simulink model "Test2_2"  (R2021a)
(part 1 of 3)
settings: Solver=FixedStepAuto  StartTime=0  StopTime=0.2  FixedStep=0.2  RelTol=1e-3
libraries: spsDistributedParametersLineLib x212, spsThreePhaseSeriesRLCLoadLib x70, spsThreePhaseVIMeasurementLib x8, spsGroundLib x1, spsThreePhaseSourceLib x1, spsSeriesRLCBranchLib x1, spspowerguiLib x1
settings Model: Creator=Admin  LastModifiedBy=Admin

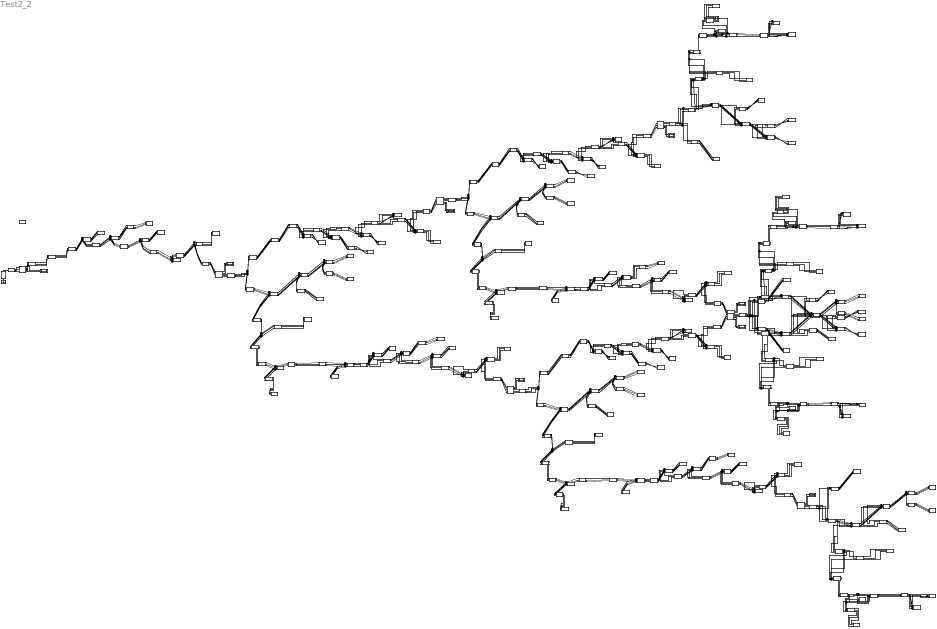
== system Test2_2 ==
  Ground : spsGroundLib/Ground  LConnTagsString=a
  Line 1 : spsDistributedParametersLineLib/Distributed Parameters Line  Phases=3  Length=1.11  Frequency=50  Resistance=[0.502970710632245 0.0486237908083191 0.0486712220507153;0.0486237908083191 0.502875844822084 0.0486237934466192;0.0486712220507153 0.0486237934466192 0.502970710632245]  Inductance=[0.00286900545038753 0.00133270803418135 0.00132951476746136;0.00133270803418135 0.00286931445999602 0.00133799988507366;0.00132951476746136 0.00133799988507366 0.00286900545038753]  Capacitance=[8.11484299003193e-09 -1.94249816214699e-09 -1.86930692621136e-09;-1.94249816214699e-09 8.0425699231653e-09 -1.98049571960044e-09;-1.86930692621136e-09 -1.98049571960044e-09 8.13337738722527e-09]  x1=[235.740627449821 9842.13785797111 9841.50657979125;314.159265358979 314.159265358979 314.159265358979;1.08127877463144 2.25146816148109 -2.46064601505037]  x2=[235.740963564487 9842.14706191756 9841.51580387368;314.159265358979 314.159265358979 314.159265358979;1.08127828242004 2.25146728367899 -2.46064690041362]  x3=[0.20667213359049 25.036273858011 25.2268910022424;314.159265358979 314.159265358979 314.159265358979;1.079589872229 2.25010012848936 -2.46201559089723]  x4=[0.206672133614643 25.0362738655198 25.2268910099133;314.159265358979 314.159265358979 314.159265358979;1.08127828238506 2.25146728367861 -2.46064690041429]  x5=5.37516004033389e-06  V1=ones(3,3)  V2=ones(3,3)  I1=ones(3,3)  I2=ones(3,3)  nHarmo=1  Measurements=None  Decoupling=off  VsMag0=0  VrMag0=0  VsAngle0=0  VrAngle0=0  IsMag0=0  IrMag0=0  IsAngle0=0  IrAngle0=0
      settings: SourceProductBaseCode=PS
  Line 10 : spsDistributedParametersLineLib/Distributed Parameters Line  Phases=3  Length=0.02  Frequency=50  Resistance=[0.646656091154803 0.0486237908083191 0.0486712220507153;0.0486237908083191 0.646561225344642 0.0486237934466192;0.0486712220507153 0.0486237934466192 0.646656091154803]  Inductance=[0.00282448912315926 0.00133270803418135 0.00132951476746136;0.00133270803418135 0.00282479813276775 0.00133799988507366;0.00132951476746136 0.00133799988507366 0.00282448912315926]  Capacitance=[7.89543174552926e-09 -1.85986777702161e-09 -1.7901190036642e-09;-1.85986777702161e-09 7.82540023894543e-09 -1.8957321828871e-09;-1.7901190036642e-09 -1.8957321828871e-09 7.91264394645417e-09]  x1=[131.78014733242 9843.57612220075 9843.09391339889;314.159265358979 314.159265358979 314.159265358979;1.07009614058309 2.25918230682552 -2.45295604852824]  x2=[131.780254208923 9843.54629581266 9843.0641121035;314.159265358979 314.159265358979 314.159265358979;1.07009786039608 2.25918056584775 -2.45295777590887]  x3=[0.121897583666128 22.8143812661449 23.0053055695837;314.159265358979 314.159265358979 314.159265358979;1.06824602708052 2.27345686414031 -2.43881138170621]  x4=[0.108540682306908 27.2903157642653 27.4816698646594;314.159265358979 314.159265358979 314.159265358979;1.07214379525045 2.24722551403408 -2.46482021330641]  x5=9.5829454252223e-08  V1=ones(3,3)  V2=ones(3,3)  I1=ones(3,3)  I2=ones(3,3)  nHarmo=1  Measurements=None  Decoupling=off  VsMag0=0  VrMag0=0  VsAngle0=0  VrAngle0=0  IsMag0=0  IrMag0=0  IsAngle0=0  IrAngle0=0
      settings: SourceProductBaseCode=PS
  Line 100 : spsDistributedParametersLineLib/Distributed Parameters Line  Phases=3  Length=0.12001  Frequency=50  Resistance=[0.646656091154803 0.0486237908083191 0.0486712220507153;0.0486237908083191 0.646561225344642 0.0486237934466192;0.0486712220507153 0.0486237934466192 0.646656091154803]  Inductance=[0.00282448912315926 0.00133270803418135 0.00132951476746136;0.00133270803418135 0.00282479813276775 0.00133799988507366;0.00132951476746136 0.00133799988507366 0.00282448912315926]  Capacitance=[7.89543174552926e-09 -1.85986777702161e-09 -1.7901190036642e-09;-1.85986777702161e-09 7.82540023894543e-09 -1.8957321828871e-09;-1.7901190036642e-09 -1.8957321828871e-09 7.91264394645417e-09]  x1=[132.251183868736 9822.51156326851 9822.6881155278;314.159265358979 314.159265358979 314.159265358979;1.0139776910405 -0.191624464327191 -1.76260238554906]  x2=[132.251379700384 9822.48352849832 9822.66014018258;314.159265358979 314.159265358979 314.159265358979;1.01397817548804 -0.191624813198916 -1.76260272547254]  x3=[0.116233256836359 24.7295911584912 24.9218766604658;314.159265358979 314.159265358979 314.159265358979;1.00798240761241 -0.185214983818316 -1.75624522525873]  x4=[0.115021145519369 25.2589468937937 25.4514391532114;314.159265358979 314.159265358979 314.159265358979;1.01985503692047 -0.198041980394282 -1.76896977112499]  x5=5.75024640240464e-07  V1=ones(3,3)  V2=ones(3,3)  I1=ones(3,3)  I2=ones(3,3)  nHarmo=1  Measurements=None  Decoupling=off  VsMag0=0  VrMag0=0  VsAngle0=0  VrAngle0=0  IsMag0=0  IrMag0=0  IsAngle0=0  IrAngle0=0
      settings: SourceProductBaseCode=PS
  Line 101 : spsDistributedParametersLineLib/Distributed Parameters Line  Phases=3  Length=0.82  Frequency=50  Resistance=[0.646656091154803 0.0486237908083191 0.0486712220507153;0.0486237908083191 0.646561225344642 0.0486237934466192;0.0486712220507153 0.0486237934466192 0.646656091154803]  Inductance=[0.00282448912315926 0.00133270803418135 0.00132951476746136;0.00133270803418135 0.00282479813276775 0.00133799988507366;0.00132951476746136 0.00133799988507366 0.00282448912315926]  Capacitance=[7.89543174552926e-09 -1.85986777702161e-09 -1.7901190036642e-09;-1.85986777702161e-09 7.82540023894543e-09 -1.8957321828871e-09;-1.7901190036642e-09 -1.8957321828871e-09 7.91264394645417e-09]  x1=[132.251183868736 9822.51156326851 9822.6881155278;314.159265358979 314.159265358979 314.159265358979;1.01292400621019 -0.192461547720951 -1.76344026578694]  x2=[132.254706380519 9821.98923988506 9822.16651105881;314.159265358979 314.159265358979 314.159265358979;1.01294030353769 -0.192482605604276 -1.76346112432621]  x3=[0.117790876870439 24.1120519373959 24.3038670356319;314.159265358979 314.159265358979 314.159265358979;0.99917348478268 -0.182323882366389 -1.75339911559519]  x4=[0.113404341728002 25.8369348193095 26.0292631540775;314.159265358979 314.159265358979 314.159265358979;1.02596467431606 -0.202890909757443 -1.77378526157166]  x5=3.92900762434114e-06  V1=ones(3,3)  V2=ones(3,3)  I1=ones(3,3)  I2=ones(3,3)  nHarmo=1  Measurements=None  Decoupling=off  VsMag0=0  VrMag0=0  VsAngle0=0  VrAngle0=0  IsMag0=0  IrMag0=0  IsAngle0=0  IrAngle0=0
      settings: SourceProductBaseCode=PS
  Line 102 : spsDistributedParametersLineLib/Distributed Parameters Line  Phases=3  Length=1.11  Frequency=50  Resistance=[0.646656091154803 0.0486237908083191 0.0486712220507153;0.0486237908083191 0.646561225344642 0.0486237934466192;0.0486712220507153 0.0486237934466192 0.646656091154803]  Inductance=[0.00282448912315926 0.00133270803418135 0.00132951476746136;0.00133270803418135 0.00282479813276775 0.00133799988507366;0.00132951476746136 0.00133799988507366 0.00282448912315926]  Capacitance=[7.89543174552926e-09 -1.85986777702161e-09 -1.7901190036642e-09;-1.85986777702161e-09 7.82540023894543e-09 -1.8957321828871e-09;-1.7901190036642e-09 -1.8957321828871e-09 7.91264394645417e-09]  x1=[132.22110603618 9826.55451502118 9826.72616066843;314.159265358979 314.159265358979 314.159265358979;1.01234684176435 -0.192590861949341 -1.76357146343656]  x2=[132.238781069031 9824.24966881277 9824.42365326744;314.159265358979 314.159265358979 314.159265358979;1.01243597193449 -0.192738058848091 -1.76371774540788]  x3=[0.124232108565467 21.7752977626428 21.9664339216675;314.159265358979 314.159265358979 314.159265358979;0.966849600717489 -0.177729233813201 -1.7489636968201]  x4=[0.107137659712284 28.1752500802333 28.3680257860225;314.159265358979 314.159265358979 314.159265358979;1.06340115095006 -0.205384100987335 -1.77619162891763]  x5=5.31853471099837e-06  V1=ones(3,3)  V2=ones(3,3)  I1=ones(3,3)  I2=ones(3,3)  nHarmo=1  Measurements=None  Decoupling=off  VsMag0=0  VrMag0=0  VsAngle0=0  VrAngle0=0  IsMag0=0  IrMag0=0  IsAngle0=0  IrAngle0=0
      settings: SourceProductBaseCode=PS
  Line 103 : spsDistributedParametersLineLib/Distributed Parameters Line  Phases=3  Length=0.20999  Frequency=50  Resistance=[0.646656091154803 0.0486237908083191 0.0486712220507153;0.0486237908083191 0.646561225344642 0.0486237934466192;0.0486712220507153 0.0486237934466192 0.646656091154803]  Inductance=[0.00282448912315926 0.00133270803418135 0.00132951476746136;0.00133270803418135 0.00282479813276775 0.00133799988507366;0.00132951476746136 0.00133799988507366 0.00282448912315926]  Capacitance=[7.89543174552926e-09 -1.85986777702161e-09 -1.7901190036642e-09;-1.85986777702161e-09 7.82540023894543e-09 -1.8957321828871e-09;-1.7901190036642e-09 -1.8957321828871e-09 7.91264394645417e-09]  x1=[132.22110603618 9826.55451502118 9826.72616066843;314.159265358979 314.159265358979 314.159265358979;1.01370161380985 -0.191514584537925 -1.76249416148526]  x2=[132.220703418741 9826.60479396299 9826.77613530937;314.159265358979 314.159265358979 314.159265358979;1.01370438274641 -0.191521096517127 -1.76250067247797]  x3=[0.11604976886815 25.0066881755724 25.1992168467069;314.159265358979 314.159265358979 314.159265358979;1.02480830153253 -0.212018461817681 -1.78284780104421]  x4=[0.11515209619338 25.0068429368372 25.1990818745629;314.159265358979 314.159265358979 314.159265358979;1.00219378168083 -0.171268482071947 -1.74239830051209]  x5=1.00616135492121e-06  V1=ones(3,3)  V2=ones(3,3)  I1=ones(3,3)  I2=ones(3,3)  nHarmo=1  Measurements=None  Decoupling=off  VsMag0=0  VrMag0=0  VsAngle0=0  VrAngle0=0  IsMag0=0  IrMag0=0  IsAngle0=0  IrAngle0=0
      settings: SourceProductBaseCode=PS
  Line 104 : spsDistributedParametersLineLib/Distributed Parameters Line  Phases=3  Length=0.23001  Frequency=50  Resistance=[0.476003738225748 0.351747138225748 0.351747138225748;0.351747138225748 0.476003738225748 0.351747138225748;0.351747138225748 0.351747138225748 0.476003738225748]  Inductance=[0.000705954362986426 0.000459934243504405 0.000459934243504405;0.000459934243504405 0.000705954362986426 0.000459934243504405;0.000459934243504405 0.000459934243504405 0.000705954362986426]  Capacitance=[5.7561313269996e-07 -1.37543883484145e-07 -1.37543912800485e-07;-1.37543883484145e-07 5.75613027339387e-07 -1.37543875208088e-07;-1.37543912800485e-07 -1.37543875208088e-07 5.75613005057695e-07]  x1=[4.47229783792521 9827.65587276305 9828.6527718167;314.159265358979 314.159265358979 314.159265358979;1.27259155336982 -0.110574029317674 -1.68141113561575]  x2=[4.47230354283643 9827.66037438348 9828.65727389307;314.159265358979 314.159265358979 314.159265358979;1.27258860764781 -0.110574765724932 -1.6814118720229]  x3=[0.0606364727518491 528.513670062988 528.567240688046;314.159265358979 314.159265358979 314.159265358979;1.27099282696656 -0.111531535342372 -1.68236864156729]  x4=[0.0606364726692423 528.513670156436 528.567240781746;314.159265358979 314.159265358979 314.159265358979;1.27258860804999 -0.110574765725967 -1.68141187202331]  x5=5.08421409621804e-06  V1=ones(3,3)  V2=ones(3,3)  I1=ones(3,3)  I2=ones(3,3)  nHarmo=1  Measurements=None  Decoupling=off  VsMag0=0  VrMag0=0  VsAngle0=0  VrAngle0=0  IsMag0=0  IrMag0=0  IsAngle0=0  IrAngle0=0
      settings: SourceProductBaseCode=PS
  Line 105 : spsDistributedParametersLineLib/Distributed Parameters Line  Phases=3  Length=0.28003  Frequency=50  Resistance=[0.646656091154803 0.0486237908083191 0.0486712220507153;0.0486237908083191 0.646561225344642 0.0486237934466192;0.0486712220507153 0.0486237934466192 0.646656091154803]  Inductance=[0.00282448912315926 0.00133270803418135 0.00132951476746136;0.00133270803418135 0.00282479813276775 0.00133799988507366;0.00132951476746136 0.00133799988507366 0.00282448912315926]  Capacitance=[7.89543174552926e-09 -1.85986777702161e-09 -1.7901190036642e-09;-1.85986777702161e-09 7.82540023894543e-09 -1.8957321828871e-09;-1.7901190036642e-09 -1.8957321828871e-09 7.91264394645417e-09]  x1=[131.783203312388 9842.18139381324 9841.69855997394;314.159265358979 314.159265358979 314.159265358979;1.06980400384549 2.25872965727568 -2.45340823480742]  x2=[131.783260319828 9842.18412601891 9841.70129695104;314.159265358979 314.159265358979 314.159265358979;1.06980381572691 2.25872930408743 -2.45340859096022]  x3=[0.115206681531441 25.0392814649209 25.2302987105999;314.159265358979 314.159265358979 314.159265358979;1.06856559283218 2.25773315191792 -2.45440562091191]  x4=[0.115207403330286 25.0392810388126 25.2302991433172;314.159265358979 314.159265358979 314.159265358979;1.07062067597059 2.25939089977307 -2.45274643363381]  x5=1.3417561037125e-06  V1=ones(3,3)  V2=ones(3,3)  I1=ones(3,3)  I2=ones(3,3)  nHarmo=1  Measurements=None  Decoupling=off  VsMag0=0  VrMag0=0  VsAngle0=0  VrAngle0=0  IsMag0=0  IrMag0=0  IsAngle0=0  IrAngle0=0
      settings: SourceProductBaseCode=PS
  Line 106 : spsDistributedParametersLineLib/Distributed Parameters Line  Phases=3  Length=0.24001  Frequency=50  Resistance=[0.646656091154803 0.0486237908083191 0.0486712220507153;0.0486237908083191 0.646561225344642 0.0486237934466192;0.0486712220507153 0.0486237934466192 0.646656091154803]  Inductance=[0.00282448912315926 0.00133270803418135 0.00132951476746136;0.00133270803418135 0.00282479813276775 0.00133799988507366;0.00132951476746136 0.00133799988507366 0.00282448912315926]  Capacitance=[7.89543174552926e-09 -1.85986777702161e-09 -1.7901190036642e-09;-1.85986777702161e-09 7.82540023894543e-09 -1.8957321828871e-09;-1.7901190036642e-09 -1.8957321828871e-09 7.91264394645417e-09]  x1=[132.202684239385 9826.99999536629 9827.16500331793;314.159265358979 314.159265358979 314.159265358979;1.01370346118121 -0.19151111998988 -1.76249021593862]  x2=[132.221106036175 9826.55451502137 9826.72616066862;314.159265358979 314.159265358979 314.159265358979;1.01365642513771 -0.191550483970015 -1.76253009509107]  x3=[0.126648550680777 21.7742149177941 21.9706116888815;314.159265358979 314.159265358979 314.159265358979;0.666612685174768 -0.198929797050631 -1.77234979456121]  x4=[0.120050164818543 28.2292431455141 28.4184691523611;314.159265358979 314.159265358979 314.159265358979;1.38032867226061 -0.186077938239135 -1.75515779675378]  x5=1.1500013657538e-06  V1=ones(3,3)  V2=ones(3,3)  I1=ones(3,3)  I2=ones(3,3)  nHarmo=1  Measurements=None  Decoupling=off  VsMag0=0  VrMag0=0  VsAngle0=0  VrAngle0=0  IsMag0=0  IrMag0=0  IsAngle0=0  IrAngle0=0
      settings: SourceProductBaseCode=PS
  Line 107 : spsDistributedParametersLineLib/Distributed Parameters Line  Phases=3  Length=0.03  Frequency=50  Resistance=[0.476003738225748 0.351747138225748 0.351747138225748;0.351747138225748 0.476003738225748 0.351747138225748;0.351747138225748 0.351747138225748 0.476003738225748]  Inductance=[0.000705954362986426 0.000459934243504405 0.000459934243504405;0.000459934243504405 0.000705954362986426 0.000459934243504405;0.000459934243504405 0.000459934243504405 0.000705954362986426]  Capacitance=[5.7561313269996e-07 -1.37543883484145e-07 -1.37543912800485e-07;-1.37543883484145e-07 5.75613027339387e-07 -1.37543875208088e-07;-1.37543912800485e-07 -1.37543875208088e-07 5.75613005057695e-07]  x1=[4.54470074903476 9824.69388809356 9825.69440909867;314.159265358979 314.159265358979 314.159265358979;1.2803214431057 -0.109972978030824 -1.68080889003995]  x2=[4.54470136219724 9824.6940440882 9825.69456555461;314.159265358979 314.159265358979 314.159265358979;1.28031883175789 -0.109973003530376 -1.68080891566607]  x3=[0.0616594487826835 528.884637500599 528.938393425842;314.159265358979 314.159265358979 314.159265358979;1.2755352456308 -0.110162497062282 -1.68099896514834]  x4=[0.0618747640776966 528.884574036237 528.938456879702;314.159265358979 314.159265358979 314.159265358979;1.28488039234838 -0.109908329382083 -1.68074368546453]  x5=6.63129528657629e-07  V1=ones(3,3)  V2=ones(3,3)  I1=ones(3,3)  I2=ones(3,3)  nHarmo=1  Measurements=None  Decoupling=off  VsMag0=0  VrMag0=0  VsAngle0=0  VrAngle0=0  IsMag0=0  IrMag0=0  IsAngle0=0  IrAngle0=0
      settings: SourceProductBaseCode=PS
  Line 108 : spsDistributedParametersLineLib/Distributed Parameters Line  Phases=3  Length=0.02  Frequency=50  Resistance=[0.646656091154803 0.0486237908083191 0.0486712220507153;0.0486237908083191 0.646561225344642 0.0486237934466192;0.0486712220507153 0.0486237934466192 0.646656091154803]  Inductance=[0.00282448912315926 0.00133270803418135 0.00132951476746136;0.00133270803418135 0.00282479813276775 0.00133799988507366;0.00132951476746136 0.00133799988507366 0.00282448912315926]  Capacitance=[7.89543174552926e-09 -1.85986777702161e-09 -1.7901190036642e-09;-1.85986777702161e-09 7.82540023894543e-09 -1.8957321828871e-09;-1.7901190036642e-09 -1.8957321828871e-09 7.91264394645417e-09]  x1=[132.202684239385 9826.99999536629 9827.16500331793;314.159265358979 314.159265358979 314.159265358979;1.01403463905449 -0.191248020920663 -1.76222686641772]  x2=[132.202716264605 9826.99502778241 9827.16004186565;314.159265358979 314.159265358979 314.159265358979;1.01403480645883 -0.191248234329926 -1.76222707785219]  x3=[0.116469758306098 24.6662306908165 24.8586235131847;314.159265358979 314.159265358979 314.159265358979;1.00929302677894 -0.187472612867995 -1.75848399497354]  x4=[0.114709498477322 25.3502366672254 25.5428305195539;314.159265358979 314.159265358979 314.159265358979;1.01881884545757 -0.194945364619181 -1.76589330632791]  x5=9.5829454252223e-08  V1=ones(3,3)  V2=ones(3,3)  I1=ones(3,3)  I2=ones(3,3)  nHarmo=1  Measurements=None  Decoupling=off  VsMag0=0  VrMag0=0  VsAngle0=0  VrAngle0=0  IsMag0=0  IrMag0=0  IsAngle0=0  IrAngle0=0
      settings: SourceProductBaseCode=PS
  Line 109 : spsDistributedParametersLineLib/Distributed Parameters Line  Phases=3  Length=0.5  Frequency=50  Resistance=[0.646656091154803 0.0486237908083191 0.0486712220507153;0.0486237908083191 0.646561225344642 0.0486237934466192;0.0486712220507153 0.0486237934466192 0.646656091154803]  Inductance=[0.00282448912315926 0.00133270803418135 0.00132951476746136;0.00133270803418135 0.00282479813276775 0.00133799988507366;0.00132951476746136 0.00133799988507366 0.00282448912315926]  Capacitance=[7.89543174552926e-09 -1.85986777702161e-09 -1.7901190036642e-09;-1.85986777702161e-09 7.82540023894543e-09 -1.8957321828871e-09;-1.7901190036642e-09 -1.8957321828871e-09 7.91264394645417e-09]  x1=[132.163450439569 9828.04961373003 9828.20063661273;314.159265358979 314.159265358979 314.159265358979;1.0134061317629 -0.191734356431076 -1.76271272153296]  x2=[132.202684239385 9826.99999536629 9827.16500331793;314.159265358979 314.159265358979 314.159265358979;1.01331210199175 -0.191822029162216 -1.76280142107447]  x3=[0.127642642019091 21.4277763025714 21.6237569851515;314.159265358979 314.159265358979 314.159265358979;0.663833530086098 -0.195610038536538 -1.76910978339631]  x4=[0.119417037015529 28.5638731580296 28.7529094890207;314.159265358979 314.159265358979 314.159265358979;1.38732746175765 -0.189426988396327 -1.75850389104283]  x5=2.39573635630557e-06  V1=ones(3,3)  V2=ones(3,3)  I1=ones(3,3)  I2=ones(3,3)  nHarmo=1  Measurements=None  Decoupling=off  VsMag0=0  VrMag0=0  VsAngle0=0  VrAngle0=0  IsMag0=0  IrMag0=0  IsAngle0=0  IrAngle0=0
      settings: SourceProductBaseCode=PS
  Line 11 : spsDistributedParametersLineLib/Distributed Parameters Line  Phases=3  Length=1.15  Frequency=50  Resistance=[0.646656091154803 0.0486237908083191 0.0486712220507153;0.0486237908083191 0.646561225344642 0.0486237934466192;0.0486712220507153 0.0486237934466192 0.646656091154803]  Inductance=[0.00282448912315926 0.00133270803418135 0.00132951476746136;0.00133270803418135 0.00282479813276775 0.00133799988507366;0.00132951476746136 0.00133799988507366 0.00282448912315926]  Capacitance=[7.89543174552926e-09 -1.85986777702161e-09 -1.7901190036642e-09;-1.85986777702161e-09 7.82540023894543e-09 -1.8957321828871e-09;-1.7901190036642e-09 -1.8957321828871e-09 7.91264394645417e-09]  x1=[131.78014733242 9843.57612220075 9843.09391339889;314.159265358979 314.159265358979 314.159265358979;1.06839516791455 2.25783099575686 -2.45430864594934]  x2=[131.786253662837 9842.40708440789 9841.92739858518;314.159265358979 314.159265358979 314.159265358979;1.06844505973248 2.25781032499208 -2.45432889211313]  x3=[0.119085012415456 23.8324187594584 24.02304457685;314.159265358979 314.159265358979 314.159265358979;1.05586532313826 2.2840755709886 -2.42828201401687]  x4=[0.111248251779623 26.2170755332442 26.4076419097041;314.159265358979 314.159265358979 314.159265358979;1.08006697091024 2.23264110559261 -2.47931888342463]  x5=5.51019361950282e-06  V1=ones(3,3)  V2=ones(3,3)  I1=ones(3,3)  I2=ones(3,3)  nHarmo=1  Measurements=None  Decoupling=off  VsMag0=0  VrMag0=0  VsAngle0=0  VrAngle0=0  IsMag0=0  IrMag0=0  IsAngle0=0  IrAngle0=0
      settings: SourceProductBaseCode=PS
  Line 110 : spsDistributedParametersLineLib/Distributed Parameters Line  Phases=3  Length=1.11  Frequency=50  Resistance=[0.502970710632245 0.0486237908083191 0.0486712220507153;0.0486237908083191 0.502875844822084 0.0486237934466192;0.0486712220507153 0.0486237934466192 0.502970710632245]  Inductance=[0.00286900545038753 0.00133270803418135 0.00132951476746136;0.00133270803418135 0.00286931445999602 0.00133799988507366;0.00132951476746136 0.00133799988507366 0.00286900545038753]  Capacitance=[8.11484299003193e-09 -1.94249816214699e-09 -1.86930692621136e-09;-1.94249816214699e-09 8.0425699231653e-09 -1.98049571960044e-09;-1.86930692621136e-09 -1.98049571960044e-09 8.13337738722527e-09]  x1=[235.83913417927 9836.90740881006 9836.84634716611;314.159265358979 314.159265358979 314.159265358979;0.992992288924493 -0.185705364593341 -1.75670803360608]  x2=[235.839470434418 9836.91660786522 9836.85556688069;314.159265358979 314.159265358979 314.159265358979;0.99299179671323 -0.185706242395447 -1.75670891896933]  x3=[0.206758493763478 25.022968724515 25.2149453535676;314.159265358979 314.159265358979 314.159265358979;0.991303386477297 -0.187073397587017 -1.75807760945267]  x4=[0.206758493746578 25.0229687321167 25.214945361144;314.159265358979 314.159265358979 314.159265358979;0.992991796728175 -0.185706242393996 -1.75670891897023]  x5=5.37516004033389e-06  V1=ones(3,3)  V2=ones(3,3)  I1=ones(3,3)  I2=ones(3,3)  nHarmo=1  Measurements=None  Decoupling=off  VsMag0=0  VrMag0=0  VsAngle0=0  VrAngle0=0  IsMag0=0  IrMag0=0  IsAngle0=0  IrAngle0=0
      settings: SourceProductBaseCode=PS
  Line 111 : spsDistributedParametersLineLib/Distributed Parameters Line  Phases=3  Length=0.03  Frequency=50  Resistance=[0.476003738225748 0.351747138225748 0.351747138225748;0.351747138225748 0.476003738225748 0.351747138225748;0.351747138225748 0.351747138225748 0.476003738225748]  Inductance=[0.000705954362986426 0.000459934243504405 0.000459934243504405;0.000459934243504405 0.000705954362986426 0.000459934243504405;0.000459934243504405 0.000459934243504405 0.000705954362986426]  Capacitance=[5.7561313269996e-07 -1.37543883484145e-07 -1.37543912800485e-07;-1.37543883484145e-07 5.75613027339387e-07 -1.37543875208088e-07;-1.37543912800485e-07 -1.37543875208088e-07 5.75613005057695e-07]  x1=[4.09509391274678 9837.99330493326 9838.91403693167;314.159265358979 314.159265358979 314.159265358979;1.2935600530543 -0.109040219571844 -1.67987163980105]  x2=[4.09509436601128 9837.99346113903 9838.9141935981;314.159265358979 314.159265358979 314.159265358979;1.29355716146171 -0.109040245071395 -1.67987166542717]  x3=[0.0555454320879041 529.600574024741 529.65003460435;314.159265358979 314.159265358979 314.159265358979;1.28829946804703 -0.109229738590482 -1.68006171488799]  x4=[0.0557678088405428 529.600510486855 529.650098134963;314.159265358979 314.159265358979 314.159265358979;1.29858883183727 -0.108975570935471 -1.67980643524576]  x5=6.63129528657629e-07  V1=ones(3,3)  V2=ones(3,3)  I1=ones(3,3)  I2=ones(3,3)  nHarmo=1  Measurements=None  Decoupling=off  VsMag0=0  VrMag0=0  VsAngle0=0  VrAngle0=0  IsMag0=0  IrMag0=0  IsAngle0=0  IrAngle0=0
      settings: SourceProductBaseCode=PS
  Line 112 : spsDistributedParametersLineLib/Distributed Parameters Line  Phases=3  Length=0.28003  Frequency=50  Resistance=[0.476003738225748 0.351747138225748 0.351747138225748;0.351747138225748 0.476003738225748 0.351747138225748;0.351747138225748 0.351747138225748 0.476003738225748]  Inductance=[0.000705954362986426 0.000459934243504405 0.000459934243504405;0.000459934243504405 0.000705954362986426 0.000459934243504405;0.000459934243504405 0.000459934243504405 0.000705954362986426]  Capacitance=[5.7561313269996e-07 -1.37543883484145e-07 -1.37543912800485e-07;-1.37543883484145e-07 5.75613027339387e-07 -1.37543875208088e-07;-1.37543912800485e-07 -1.37543875208088e-07 5.75613005057695e-07]  x1=[4.09509391274678 9837.99330493326 9838.91403693167;314.159265358979 314.159265358979 314.159265358979;1.29182377567967 -0.110080666377091 -1.68091208652586]  x2=[4.09504726943923 9837.69896048846 9838.62067548761;314.159265358979 314.159265358979 314.159265358979;1.28807724990493 -0.110095919504453 -1.68092754802377]  x3=[0.0547281253877361 520.910739259854 520.95393370585;314.159265358979 314.159265358979 314.159265358979;0.49865318313759 -0.109359777351524 -1.68029763835162]  x4=[0.082244361651287 536.94771402624 537.003359247534;314.159265358979 314.159265358979 314.159265358979;1.78149310040174 -0.111943471076262 -1.68267181039533]  x5=6.18987206366653e-06  V1=ones(3,3)  V2=ones(3,3)  I1=ones(3,3)  I2=ones(3,3)  nHarmo=1  Measurements=None  Decoupling=off  VsMag0=0  VrMag0=0  VsAngle0=0  VrAngle0=0  IsMag0=0  IrMag0=0  IsAngle0=0  IrAngle0=0
      settings: SourceProductBaseCode=PS
  Line 113 : spsDistributedParametersLineLib/Distributed Parameters Line  Phases=3  Length=0.28003  Frequency=50  Resistance=[0.646656091154803 0.0486237908083191 0.0486712220507153;0.0486237908083191 0.646561225344642 0.0486237934466192;0.0486712220507153 0.0486237934466192 0.646656091154803]  Inductance=[0.00282448912315926 0.00133270803418135 0.00132951476746136;0.00133270803418135 0.00282479813276775 0.00133799988507366;0.00132951476746136 0.00133799988507366 0.00282448912315926]  Capacitance=[7.89543174552926e-09 -1.85986777702161e-09 -1.7901190036642e-09;-1.85986777702161e-09 7.82540023894543e-09 -1.8957321828871e-09;-1.7901190036642e-09 -1.8957321828871e-09 7.91264394645417e-09]  x1=[131.969774279842 9836.6504997016 9836.73739163194;314.159265358979 314.159265358979 314.159265358979;1.01399588860223 -0.190917998076078 -1.76189341770976]  x2=[131.99796100534 9835.17324620966 9835.2691044748;314.159265358979 314.159265358979 314.159265358979;1.01397276776253 -0.191008554452366 -1.76198420642346]  x3=[0.141073246705685 17.0169663215439 17.2079022231078;314.159265358979 314.159265358979 314.159265358979;0.63939633992786 -0.132458922535815 -1.70742412031073]  x4=[0.112046147843418 33.0740086276995 33.262489789006;314.159265358979 314.159265358979 314.159265358979;1.4922539386786 -0.221305323744142 -1.79038525061112]  x5=1.3417561037125e-06  V1=ones(3,3)  V2=ones(3,3)  I1=ones(3,3)  I2=ones(3,3)  nHarmo=1  Measurements=None  Decoupling=off  VsMag0=0  VrMag0=0  VsAngle0=0  VrAngle0=0  IsMag0=0  IrMag0=0  IsAngle0=0  IrAngle0=0
      settings: SourceProductBaseCode=PS
  Line 114 : spsDistributedParametersLineLib/Distributed Parameters Line  Phases=3  Length=0.3  Frequency=50  Resistance=[0.80718830189013 0.0486237908083191 0.0486712220507153;0.0486237908083191 0.807093436079969 0.0486237934466192;0.0486712220507153 0.0486237934466192 0.80718830189013]  Inductance=[0.00279786707424938 0.00133270803418135 0.00132951476746136;0.00133270803418135 0.00279817608385787 0.00133799988507366;0.00132951476746136 0.00133799988507366 0.00279786707424938]  Capacitance=[7.73340098830622e-09 -1.79942827973291e-09 -1.73218055098733e-09;-1.79942827973291e-09 7.66505189233746e-09 -1.83375898618858e-09;-1.73218055098733e-09 -1.83375898618858e-09 7.749673531177e-09]  x1=[55.2881000392909 9835.25797331996 9835.43293630037;314.159265358979 314.159265358979 314.159265358979;1.0796782128636 -0.195337139904711 -1.76627292103014]  x2=[55.2881055931467 9835.25858087199 9835.43354489027;314.159265358979 314.159265358979 314.159265358979;1.07967815994283 -0.195337241403251 -1.76627302337392]  x3=[0.0481731421242871 24.9554512932554 25.1460380670562;314.159265358979 314.159265358979 314.159265358979;1.07922996125495 -0.195688681371146 -1.76662475988699]  x4=[0.0481731421014888 24.9554512934377 25.1460380672614;314.159265358979 314.159265358979 314.159265358979;1.07967816011044 -0.195337241403375 -1.76627302337436]  x5=1.42674452918375e-06  V1=ones(3,3)  V2=ones(3,3)  I1=ones(3,3)  I2=ones(3,3)  nHarmo=1  Measurements=None  Decoupling=off  VsMag0=0  VrMag0=0  VsAngle0=0  VrAngle0=0  IsMag0=0  IrMag0=0  IsAngle0=0  IrAngle0=0
      settings: SourceProductBaseCode=PS
  Line 115 : spsDistributedParametersLineLib/Distributed Parameters Line  Phases=3  Length=0.25999  Frequency=50  Resistance=[0.646656091154803 0.0486237908083191 0.0486712220507153;0.0486237908083191 0.646561225344642 0.0486237934466192;0.0486712220507153 0.0486237934466192 0.646656091154803]  Inductance=[0.00282448912315926 0.00133270803418135 0.00132951476746136;0.00133270803418135 0.00282479813276775 0.00133799988507366;0.00132951476746136 0.00133799988507366 0.00282448912315926]  Capacitance=[7.89543174552926e-09 -1.85986777702161e-09 -1.7901190036642e-09;-1.85986777702161e-09 7.82540023894543e-09 -1.8957321828871e-09;-1.7901190036642e-09 -1.8957321828871e-09 7.91264394645417e-09]  x1=[131.99796100534 9835.17324620966 9835.2691044748;314.159265358979 314.159265358979 314.159265358979;1.0140029336849 -0.190984589608281 -1.76196021876654]  x2=[132.024087588405 9833.79972311698 9833.90390262215;314.159265358979 314.159265358979 314.159265358979;1.01398161532232 -0.191068423345733 -1.76204426590704]  x3=[0.141062318523068 17.0145420908718 17.2054261259926;314.159265358979 314.159265358979 314.159265358979;0.640117650918494 -0.131549162527091 -1.70651762702353]  x4=[0.112023360712419 33.0717803135698 33.2602351475184;314.159265358979 314.159265358979 314.159265358979;1.49142043019661 -0.221848078375874 -1.79092951297781]  x5=1.24573499055177e-06  V1=ones(3,3)  V2=ones(3,3)  I1=ones(3,3)  I2=ones(3,3)  nHarmo=1  Measurements=None  Decoupling=off  VsMag0=0  VrMag0=0  VsAngle0=0  VrAngle0=0  IsMag0=0  IrMag0=0  IsAngle0=0  IrAngle0=0
      settings: SourceProductBaseCode=PS
  Line 116 : spsDistributedParametersLineLib/Distributed Parameters Line  Phases=3  Length=0.3  Frequency=50  Resistance=[0.80718830189013 0.0486237908083191 0.0486712220507153;0.0486237908083191 0.807093436079969 0.0486237934466192;0.0486712220507153 0.0486237934466192 0.80718830189013]  Inductance=[0.00279786707424938 0.00133270803418135 0.00132951476746136;0.00133270803418135 0.00279817608385787 0.00133799988507366;0.00132951476746136 0.00133799988507366 0.00279786707424938]  Capacitance=[7.73340098830622e-09 -1.79942827973291e-09 -1.73218055098733e-09;-1.79942827973291e-09 7.66505189233746e-09 -1.83375898618858e-09;-1.73218055098733e-09 -1.83375898618858e-09 7.749673531177e-09]  x1=[54.9043263508303 9842.26811697933 9841.86526506277;314.159265358979 314.159265358979 314.159265358979;1.02620626264612 2.26302453435807 -2.44915226876805]  x2=[54.9043318661299 9842.26872496441 9841.86587405069;314.159265358979 314.159265358979 314.159265358979;1.02620620972537 2.26302443285953 -2.44915237111184]  x3=[0.047838755795002 24.9732384524023 25.1624834624731;314.159265358979 314.159265358979 314.159265358979;1.02575801108249 2.26267299289159 -2.44950410762541]  x4=[0.0478387557778777 24.9732384525614 25.1624834627157;314.159265358979 314.159265358979 314.159265358979;1.02620620975078 2.26302443285979 -2.44915237111201]  x5=1.42674452918375e-06  V1=ones(3,3)  V2=ones(3,3)  I1=ones(3,3)  I2=ones(3,3)  nHarmo=1  Measurements=None  Decoupling=off  VsMag0=0  VrMag0=0  VsAngle0=0  VrAngle0=0  IsMag0=0  IrMag0=0  IsAngle0=0  IrAngle0=0
      settings: SourceProductBaseCode=PS
  Line 117 : spsDistributedParametersLineLib/Distributed Parameters Line  Phases=3  Length=0.02  Frequency=50  Resistance=[0.476003738225748 0.351747138225748 0.351747138225748;0.351747138225748 0.476003738225748 0.351747138225748;0.351747138225748 0.351747138225748 0.476003738225748]  Inductance=[0.000705954362986426 0.000459934243504405 0.000459934243504405;0.000459934243504405 0.000705954362986426 0.000459934243504405;0.000459934243504405 0.000459934243504405 0.000705954362986426]  Capacitance=[5.7561313269996e-07 -1.37543883484145e-07 -1.37543912800485e-07;-1.37543883484145e-07 5.75613027339387e-07 -1.37543875208088e-07;-1.37543912800485e-07 -1.37543875208088e-07 5.75613005057695e-07]  x1=[4.09509849376777 9838.01791398499 9838.93857581749;314.159265358979 314.159265358979 314.159265358979;1.2938993673486 -0.108997253073943 -1.67982865834034]  x2=[4.09509391274678 9837.99330493326 9838.91403693167;314.159265358979 314.159265358979 314.159265358979;1.29362949581615 -0.10899860669318 -1.6798300269256]  x3=[0.055008558850981 520.086041396904 520.129066709848;314.159265358979 314.159265358979 314.159265358979;0.496136253846119 -0.107929377975014 -1.6788680477037]  x4=[0.0828539719056332 539.170125558804 539.226033809142;314.159265358979 314.159265358979 314.159265358979;1.78881551595223 -0.110110415660987 -1.68083834754062]  x5=4.42086352438419e-07  V1=ones(3,3)  V2=ones(3,3)  I1=ones(3,3)  I2=ones(3,3)  nHarmo=1  Measurements=None  Decoupling=off  VsMag0=0  VrMag0=0  VsAngle0=0  VrAngle0=0  IsMag0=0  IrMag0=0  IsAngle0=0  IrAngle0=0
      settings: SourceProductBaseCode=PS
  Line 118 : spsDistributedParametersLineLib/Distributed Parameters Line  Phases=3  Length=1.7101  Frequency=50  Resistance=[0.646656091154803 0.0486237908083191 0.0486712220507153;0.0486237908083191 0.646561225344642 0.0486237934466192;0.0486712220507153 0.0486237934466192 0.646656091154803]  Inductance=[0.00282448912315926 0.00133270803418135 0.00132951476746136;0.00133270803418135 0.00282479813276775 0.00133799988507366;0.00132951476746136 0.00133799988507366 0.00282448912315926]  Capacitance=[7.89543174552926e-09 -1.85986777702161e-09 -1.7901190036642e-09;-1.85986777702161e-09 7.82540023894543e-09 -1.8957321828871e-09;-1.7901190036642e-09 -1.8957321828871e-09 7.91264394645417e-09]  x1=[131.78963435106 9847.162216281 9847.19454867017;314.159265358979 314.159265358979 314.159265358979;1.01202388392922 -0.191887458432444 -1.76286358346047]  x2=[131.969468815274 9836.96956151981 9837.05506258634;314.159265358979 314.159265358979 314.159265358979;1.01197903729776 -0.192611530578667 -1.76358837211047]  x3=[0.145389877456535 15.4833105634543 15.6751642135649;314.159265358979 314.159265358979 314.159265358979;0.643659639736105 -0.158806929059593 -1.73392719813837]  x4=[0.108136878891712 34.5263356371296 34.7151876789957;314.159265358979 314.159265358979 314.159265358979;1.51421717010998 -0.208726092984649 -1.77794009585278]  x5=8.19389748583632e-06  V1=ones(3,3)  V2=ones(3,3)  I1=ones(3,3)  I2=ones(3,3)  nHarmo=1  Measurements=None  Decoupling=off  VsMag0=0  VrMag0=0  VsAngle0=0  VrAngle0=0  IsMag0=0  IrMag0=0  IsAngle0=0  IrAngle0=0
      settings: SourceProductBaseCode=PS
  Line 119 : spsDistributedParametersLineLib/Distributed Parameters Line  Phases=3  Length=0.02  Frequency=50  Resistance=[0.646656091154803 0.0486237908083191 0.0486712220507153;0.0486237908083191 0.646561225344642 0.0486237934466192;0.0486712220507153 0.0486237934466192 0.646656091154803]  Inductance=[0.00282448912315926 0.00133270803418135 0.00132951476746136;0.00133270803418135 0.00282479813276775 0.00133799988507366;0.00132951476746136 0.00133799988507366 0.00282448912315926]  Capacitance=[7.89543174552926e-09 -1.85986777702161e-09 -1.7901190036642e-09;-1.85986777702161e-09 7.82540023894543e-09 -1.8957321828871e-09;-1.7901190036642e-09 -1.8957321828871e-09 7.91264394645417e-09]  x1=[131.78963435106 9847.162216281 9847.19454867017;314.159265358979 314.159265358979 314.159265358979;1.01456796703285 -0.189866351496926 -1.76084055257426]  x2=[131.789708123298 9847.15084443322 9847.1831921629;314.159265358979 314.159265358979 314.159265358979;1.01456833036841 -0.189866797279933 -1.76084099394437]  x3=[0.117186036599485 24.2942819333447 24.4865980251452;314.159265358979 314.159265358979 314.159265358979;1.00345222744801 -0.18020041704083 -1.7512577172572]  x4=[0.113283043231375 25.8266470199092 26.0194083604586;314.159265358979 314.159265358979 314.159265358979;1.02603644384263 -0.198982403670526 -1.76988250781932]  x5=9.5829454252223e-08  V1=ones(3,3)  V2=ones(3,3)  I1=ones(3,3)  I2=ones(3,3)  nHarmo=1  Measurements=None  Decoupling=off  VsMag0=0  VrMag0=0  VsAngle0=0  VrAngle0=0  IsMag0=0  IrMag0=0  IsAngle0=0  IrAngle0=0
      settings: SourceProductBaseCode=PS
  Line 12 : spsDistributedParametersLineLib/Distributed Parameters Line  Phases=3  Length=0.18999  Frequency=50  Resistance=[0.646656091154803 0.0486237908083191 0.0486712220507153;0.0486237908083191 0.646561225344642 0.0486237934466192;0.0486712220507153 0.0486237934466192 0.646656091154803]  Inductance=[0.00282448912315926 0.00133270803418135 0.00132951476746136;0.00133270803418135 0.00282479813276775 0.00133799988507366;0.00132951476746136 0.00133799988507366 0.00282448912315926]  Capacitance=[7.89543174552926e-09 -1.85986777702161e-09 -1.7901190036642e-09;-1.85986777702161e-09 7.82540023894543e-09 -1.8957321828871e-09;-1.7901190036642e-09 -1.8957321828871e-09 7.91264394645417e-09]  x1=[131.786253662837 9842.40708440789 9841.92739858518;314.159265358979 314.159265358979 314.159265358979;1.06989014891082 2.25895835343369 -2.45317977082974]  x2=[131.786489596904 9842.35119376625 9841.8716084111;314.159265358979 314.159265358979 314.159265358979;1.06989273919799 2.25895711321375 -2.45318098871556]  x3=[0.116357118798103 24.6866847362085 24.8777465249464;314.159265358979 314.159265358979 314.159265358979;1.06778314228593 2.26583494760056 -2.44635281242686]  x4=[0.11407288640751 25.399194553097 25.5902625631328;314.159265358979 314.159265358979 314.159265358979;1.07175310159526 2.25204941579955 -2.46004210872937]  x5=9.10331900668992e-07  V1=ones(3,3)  V2=ones(3,3)  I1=ones(3,3)  I2=ones(3,3)  nHarmo=1  Measurements=None  Decoupling=off  VsMag0=0  VrMag0=0  VsAngle0=0  VrAngle0=0  IsMag0=0  IrMag0=0  IsAngle0=0  IrAngle0=0
      settings: SourceProductBaseCode=PS
  Line 120 : spsDistributedParametersLineLib/Distributed Parameters Line  Phases=3  Length=0.02  Frequency=50  Resistance=[0.646656091154803 0.0486237908083191 0.0486712220507153;0.0486237908083191 0.646561225344642 0.0486237934466192;0.0486712220507153 0.0486237934466192 0.646656091154803]  Inductance=[0.00282448912315926 0.00133270803418135 0.00132951476746136;0.00133270803418135 0.00282479813276775 0.00133799988507366;0.00132951476746136 0.00133799988507366 0.00282448912315926]  Capacitance=[7.89543174552926e-09 -1.85986777702161e-09 -1.7901190036642e-09;-1.85986777702161e-09 7.82540023894543e-09 -1.8957321828871e-09;-1.7901190036642e-09 -1.8957321828871e-09 7.91264394645417e-09]  x1=[131.787452147845 9847.29257777326 9847.32427259302;314.159265358979 314.159265358979 314.159265358979;1.01456814601826 -0.189857414577419 -1.76083161138094]  x2=[131.78963435106 9847.162216281 9847.19454867017;314.159265358979 314.159265358979 314.159265358979;1.01456796703285 -0.189866351496926 -1.76084055257426]  x3=[0.14778921749857 14.7638726634964 14.9549908371047;314.159265358979 314.159265358979 314.159265358979;0.64278692680858 -0.139234054200145 -1.71479444155034]  x4=[0.107174848603431 35.3820281836619 35.5717093262689;314.159265358979 314.159265358979 314.159265358979;1.53921547705784 -0.210996866173907 -1.78020418899243]  x5=9.5829454252223e-08  V1=ones(3,3)  V2=ones(3,3)  I1=ones(3,3)  I2=ones(3,3)  nHarmo=1  Measurements=None  Decoupling=off  VsMag0=0  VrMag0=0  VsAngle0=0  VrAngle0=0  IsMag0=0  IrMag0=0  IsAngle0=0  IrAngle0=0
      settings: SourceProductBaseCode=PS
  Line 121 : spsDistributedParametersLineLib/Distributed Parameters Line  Phases=3  Length=1.15  Frequency=50  Resistance=[0.646656091154803 0.0486237908083191 0.0486712220507153;0.0486237908083191 0.646561225344642 0.0486237934466192;0.0486712220507153 0.0486237934466192 0.646656091154803]  Inductance=[0.00282448912315926 0.00133270803418135 0.00132951476746136;0.00133270803418135 0.00282479813276775 0.00133799988507366;0.00132951476746136 0.00133799988507366 0.00282448912315926]  Capacitance=[7.89543174552926e-09 -1.85986777702161e-09 -1.7901190036642e-09;-1.85986777702161e-09 7.82540023894543e-09 -1.8957321828871e-09;-1.7901190036642e-09 -1.8957321828871e-09 7.91264394645417e-09]  x1=[131.787452147845 9847.29257777326 9847.32427259302;314.159265358979 314.159265358979 314.159265358979;1.01286717334972 -0.191208725646075 -1.76218420880204]  x2=[131.795124099996 9846.30754125141 9846.34138792809;314.159265358979 314.159265358979 314.159265358979;1.01288407572261 -0.191227572528419 -1.76220275886342]  x3=[0.117555927241626 24.0170117520535 24.2086408048522;314.159265358979 314.159265358979 314.159265358979;0.987712185427898 -0.169907877400456 -1.74108718091504]  x4=[0.112845475747904 26.0464980292633 26.2388559876714;314.159265358979 314.159265358979 314.159265358979;1.03732212319896 -0.212189953781318 -1.78299032794862]  x5=5.51019361950282e-06  V1=ones(3,3)  V2=ones(3,3)  I1=ones(3,3)  I2=ones(3,3)  nHarmo=1  Measurements=None  Decoupling=off  VsMag0=0  VrMag0=0  VsAngle0=0  VrAngle0=0  IsMag0=0  IrMag0=0  IsAngle0=0  IrAngle0=0
      settings: SourceProductBaseCode=PS
  Line 122 : spsDistributedParametersLineLib/Distributed Parameters Line  Phases=3  Length=0.18999  Frequency=50  Resistance=[0.646656091154803 0.0486237908083191 0.0486712220507153;0.0486237908083191 0.646561225344642 0.0486237934466192;0.0486712220507153 0.0486237934466192 0.646656091154803]  Inductance=[0.00282448912315926 0.00133270803418135 0.00132951476746136;0.00133270803418135 0.00282479813276775 0.00133799988507366;0.00132951476746136 0.00133799988507366 0.00282448912315926]  Capacitance=[7.89543174552926e-09 -1.85986777702161e-09 -1.7901190036642e-09;-1.85986777702161e-09 7.82540023894543e-09 -1.8957321828871e-09;-1.7901190036642e-09 -1.8957321828871e-09 7.91264394645417e-09]  x1=[131.795124099996 9846.30754125141 9846.34138792809;314.159265358979 314.159265358979 314.159265358979;1.01432916490095 -0.190079544086808 -1.76105363758003]  x2=[131.795597782904 9846.23965531491 9846.27364581802;314.159265358979 314.159265358979 314.159265358979;1.01433036591315 -0.190080426279994 -1.76105449806968]  x3=[0.116161842520844 24.6469824819463 24.8392822352376;314.159265358979 314.159265358979 314.159265358979;1.00519081246749 -0.180333278967887 -1.7513874762438]  x4=[0.114292904131207 25.4598829486549 25.6524864091078;314.159265358979 314.159265358979 314.159265358979;1.02332982794793 -0.199739070909157 -1.77063803893718]  x5=9.10331900668992e-07  V1=ones(3,3)  V2=ones(3,3)  I1=ones(3,3)  I2=ones(3,3)  nHarmo=1  Measurements=None  Decoupling=off  VsMag0=0  VrMag0=0  VsAngle0=0  VrAngle0=0  IsMag0=0  IrMag0=0  IsAngle0=0  IrAngle0=0
      settings: SourceProductBaseCode=PS
  Line 123 : spsDistributedParametersLineLib/Distributed Parameters Line  Phases=3  Length=0.34002  Frequency=50  Resistance=[0.646656091154803 0.0486237908083191 0.0486712220507153;0.0486237908083191 0.646561225344642 0.0486237934466192;0.0486712220507153 0.0486237934466192 0.646656091154803]  Inductance=[0.00282448912315926 0.00133270803418135 0.00132951476746136;0.00133270803418135 0.00282479813276775 0.00133799988507366;0.00132951476746136 0.00133799988507366 0.00282448912315926]  Capacitance=[7.89543174552926e-09 -1.85986777702161e-09 -1.7901190036642e-09;-1.85986777702161e-09 7.82540023894543e-09 -1.8957321828871e-09;-1.7901190036642e-09 -1.8957321828871e-09 7.91264394645417e-09]  x1=[131.795124099996 9846.30754125141 9846.34138792809;314.159265358979 314.159265358979 314.159265358979;1.01410332691028 -0.190258957537808 -1.76123322181993]  x2=[131.79645943779 9846.13376830013 9846.16798612067;314.159265358979 314.159265358979 314.159265358979;1.01410645377202 -0.190262432091065 -1.76123664304613]  x3=[0.116649255619361 24.4399610843963 24.6321166394377;314.159265358979 314.159265358979 314.159265358979;0.999557395557013 -0.177733718740891 -1.7488234019682]  x4=[0.113804063026815 25.6595672305769 25.8521632491326;314.159265358979 314.159265358979 314.159265358979;1.02849785555148 -0.202589231127301 -1.77345814161857]  x5=1.62919655174204e-06  V1=ones(3,3)  V2=ones(3,3)  I1=ones(3,3)  I2=ones(3,3)  nHarmo=1  Measurements=None  Decoupling=off  VsMag0=0  VrMag0=0  VsAngle0=0  VrAngle0=0  IsMag0=0  IrMag0=0  IsAngle0=0  IrAngle0=0
      settings: SourceProductBaseCode=PS
  Line 124 : spsDistributedParametersLineLib/Distributed Parameters Line  Phases=3  Length=0.12001  Frequency=50  Resistance=[0.646656091154803 0.0486237908083191 0.0486712220507153;0.0486237908083191 0.646561225344642 0.0486237934466192;0.0486712220507153 0.0486237934466192 0.646656091154803]  Inductance=[0.00282448912315926 0.00133270803418135 0.00132951476746136;0.00133270803418135 0.00282479813276775 0.00133799988507366;0.00132951476746136 0.00133799988507366 0.00282448912315926]  Capacitance=[7.89543174552926e-09 -1.85986777702161e-09 -1.7901190036642e-09;-1.85986777702161e-09 7.82540023894543e-09 -1.8957321828871e-09;-1.7901190036642e-09 -1.8957321828871e-09 7.91264394645417e-09]  x1=[131.79645943779 9846.13376830013 9846.16798612067;314.159265358979 314.159265358979 314.159265358979;1.01443763164529 -0.189999333021849 -1.76097329352523]  x2=[131.796616681841 9846.11151418436 9846.14578202988;314.159265358979 314.159265358979 314.159265358979;1.01443797218558 -0.189999525698642 -1.76097347934481]  x3=[0.115688822514334 24.8496987880735 25.0421056368795;314.159265358979 314.159265358979 314.159265358979;1.00948373628436 -0.184665785682116 -1.75568319606813]  x4=[0.114769102781434 25.2587615645484 25.4513284312002;314.159265358979 314.159265358979 314.159265358979;1.01925019127265 -0.19538905287422 -1.76632101925296]  x5=5.75024640240464e-07  V1=ones(3,3)  V2=ones(3,3)  I1=ones(3,3)  I2=ones(3,3)  nHarmo=1  Measurements=None  Decoupling=off  VsMag0=0  VrMag0=0  VsAngle0=0  VrAngle0=0  IsMag0=0  IrMag0=0  IsAngle0=0  IrAngle0=0
      settings: SourceProductBaseCode=PS
  Line 125 : spsDistributedParametersLineLib/Distributed Parameters Line  Phases=3  Length=0.82  Frequency=50  Resistance=[0.646656091154803 0.0486237908083191 0.0486712220507153;0.0486237908083191 0.646561225344642 0.0486237934466192;0.0486712220507153 0.0486237934466192 0.646656091154803]  Inductance=[0.00282448912315926 0.00133270803418135 0.00132951476746136;0.00133270803418135 0.00282479813276775 0.00133799988507366;0.00132951476746136 0.00133799988507366 0.00282448912315926]  Capacitance=[7.89543174552926e-09 -1.85986777702161e-09 -1.7901190036642e-09;-1.85986777702161e-09 7.82540023894543e-09 -1.8957321828871e-09;-1.7901190036642e-09 -1.8957321828871e-09 7.91264394645417e-09]  x1=[131.79645943779 9846.13376830013 9846.16798612067;314.159265358979 314.159265358979 314.159265358979;1.01338394681498 -0.190836416415608 -1.76181117376311]  x2=[131.798448633159 9845.85936133177 9845.89411829139;314.159265358979 314.159265358979 314.159265358979;1.01338967345748 -0.190842524652357 -1.7618171921642]  x3=[0.116156034640599 24.6292386412461 24.8212767515323;314.159265358979 314.159265358979 314.159265358979;1.00421933065038 -0.183377286388867 -1.75442129343352]  x4=[0.114230826143699 25.43939280888 25.631706637913;314.159265358979 314.159265358979 314.159265358979;1.02146389761526 -0.199029289615306 -1.76993963449896]  x5=3.92900762434114e-06  V1=ones(3,3)  V2=ones(3,3)  I1=ones(3,3)  I2=ones(3,3)  nHarmo=1  Measurements=None  Decoupling=off  VsMag0=0  VrMag0=0  VsAngle0=0  VrAngle0=0  IsMag0=0  IrMag0=0  IsAngle0=0  IrAngle0=0
      settings: SourceProductBaseCode=PS
  Line 126 : spsDistributedParametersLineLib/Distributed Parameters Line  Phases=3  Length=1.11  Frequency=50  Resistance=[0.646656091154803 0.0486237908083191 0.0486712220507153;0.0486237908083191 0.646561225344642 0.0486237934466192;0.0486712220507153 0.0486237934466192 0.646656091154803]  Inductance=[0.00282448912315926 0.00133270803418135 0.00132951476746136;0.00133270803418135 0.00282479813276775 0.00133799988507366;0.00132951476746136 0.00133799988507366 0.00282448912315926]  Capacitance=[7.89543174552926e-09 -1.85986777702161e-09 -1.7901190036642e-09;-1.85986777702161e-09 7.82540023894543e-09 -1.8957321828871e-09;-1.7901190036642e-09 -1.8957321828871e-09 7.91264394645417e-09]  x1=[131.658556977053 9855.46192679251 9855.45612531466;314.159265358979 314.159265358979 314.159265358979;1.01292223444942 -0.190644835208617 -1.76162030059823]  x2=[131.787452147845 9847.29257777326 9847.32427259302;314.159265358979 314.159265358979 314.159265358979;1.01292738477161 -0.191160891625946 -1.76213632924731]  x3=[0.150968110922885 13.7829298562887 13.9704578808499;314.159265358979 314.159265358979 314.159265358979;0.627058398376765 -0.101240690932242 -1.67772512052392]  x4=[0.10662672513911 36.3724026603085 36.5610287452261;314.159265358979 314.159265358979 314.159265358979;1.57278809680062 -0.225754949119496 -1.7949196071371]  x5=5.31853471099837e-06  V1=ones(3,3)  V2=ones(3,3)  I1=ones(3,3)  I2=ones(3,3)  nHarmo=1  Measurements=None  Decoupling=off  VsMag0=0  VrMag0=0  VsAngle0=0  VrAngle0=0  IsMag0=0  IrMag0=0  IsAngle0=0  IrAngle0=0
      settings: SourceProductBaseCode=PS
  Line 127 : spsDistributedParametersLineLib/Distributed Parameters Line  Phases=3  Length=0.26  Frequency=50  Resistance=[0.646656091154803 0.0486237908083191 0.0486712220507153;0.0486237908083191 0.646561225344642 0.0486237934466192;0.0486712220507153 0.0486237934466192 0.646656091154803]  Inductance=[0.00282448912315926 0.00133270803418135 0.00132951476746136;0.00133270803418135 0.00282479813276775 0.00133799988507366;0.00132951476746136 0.00133799988507366 0.00282448912315926]  Capacitance=[7.89543174552926e-09 -1.85986777702161e-09 -1.7901190036642e-09;-1.85986777702161e-09 7.82540023894543e-09 -1.8957321828871e-09;-1.7901190036642e-09 -1.8957321828871e-09 7.91264394645417e-09]  x1=[131.783260319828 9842.18412601891 9841.70129695103;314.159265358979 314.159265358979 314.159265358979;1.06983396659643 2.25875325697301 -2.45338461527319]  x2=[131.783270412709 9842.18460175048 9841.70177356538;314.159265358979 314.159265358979 314.159265358979;1.06983393356834 2.25875319547459 -2.45338467729194]  x3=[0.115208136297893 25.0398492860678 25.2308756133217;314.159265358979 314.159265358979 314.159265358979;1.06944257571588 2.25844230509264 -2.45369586338781]  x4=[0.115208136255793 25.0398492861385 25.230875613471;314.159265358979 314.159265358979 314.159265358979;1.06983393364077 2.2587531954749 -2.45338467729245]  x5=1.2457829052789e-06  V1=ones(3,3)  V2=ones(3,3)  I1=ones(3,3)  I2=ones(3,3)  nHarmo=1  Measurements=None  Decoupling=off  VsMag0=0  VrMag0=0  VsAngle0=0  VrAngle0=0  IsMag0=0  IrMag0=0  IsAngle0=0  IrAngle0=0
      settings: SourceProductBaseCode=PS
  Line 128 : spsDistributedParametersLineLib/Distributed Parameters Line  Phases=3  Length=0.20999  Frequency=50  Resistance=[0.646656091154803 0.0486237908083191 0.0486712220507153;0.0486237908083191 0.646561225344642 0.0486237934466192;0.0486712220507153 0.0486237934466192 0.646656091154803]  Inductance=[0.00282448912315926 0.00133270803418135 0.00132951476746136;0.00133270803418135 0.00282479813276775 0.00133799988507366;0.00132951476746136 0.00133799988507366 0.00282448912315926]  Capacitance=[7.89543174552926e-09 -1.85986777702161e-09 -1.7901190036642e-09;-1.85986777702161e-09 7.82540023894543e-09 -1.8957321828871e-09;-1.7901190036642e-09 -1.8957321828871e-09 7.91264394645417e-09]  x1=[131.658556977053 9855.46192679251 9855.45612531466;314.159265358979 314.159265358979 314.159265358979;1.01427700649492 -0.1895685577972 -1.76054299864693]  x2=[131.668343537696 9854.40526605829 9854.40288715582;314.159265358979 314.159265358979 314.159265358979;1.01430043736976 -0.189630277717269 -1.76060467596099]  x3=[0.133605628134306 17.553782564724 17.7390222512148;314.159265358979 314.159265358979 314.159265358979;0.865993941140582 -0.12736298451738 -1.70080941657854]  x4=[0.100032958120693 32.6461056896961 32.8424286928486;314.159265358979 314.159265358979 314.159265358979;1.21256125677002 -0.223241522073885 -1.79303397730572]  x5=1.00616135492121e-06  V1=ones(3,3)  V2=ones(3,3)  I1=ones(3,3)  I2=ones(3,3)  nHarmo=1  Measurements=None  Decoupling=off  VsMag0=0  VrMag0=0  VsAngle0=0  VrAngle0=0  IsMag0=0  IrMag0=0  IsAngle0=0  IrAngle0=0
      settings: SourceProductBaseCode=PS
  Line 129 : spsDistributedParametersLineLib/Distributed Parameters Line  Phases=3  Length=0.23002  Frequency=50  Resistance=[0.476003738225748 0.351747138225748 0.351747138225748;0.351747138225748 0.476003738225748 0.351747138225748;0.351747138225748 0.351747138225748 0.476003738225748]  Inductance=[0.000705954362986426 0.000459934243504405 0.000459934243504405;0.000459934243504405 0.000705954362986426 0.000459934243504405;0.000459934243504405 0.000459934243504405 0.000705954362986426]  Capacitance=[5.7561313269996e-07 -1.37543883484145e-07 -1.37543912800485e-07;-1.37543883484145e-07 5.75613027339387e-07 -1.37543875208088e-07;-1.37543912800485e-07 -1.37543875208088e-07 5.75613005057695e-07]  x1=[3.5476486806423 9855.45449286004 9856.29207977165;314.159265358979 314.159265358979 314.159265358979;1.29514220455488 -0.108684473617397 -1.67951382970631]  x2=[3.54709113031397 9855.21461685951 9856.05247196973;314.159265358979 314.159265358979 314.159265358979;1.29425215748696 -0.10869418572806 -1.67952364181978]  x3=[0.0430976714066817 522.46197736567 522.49809822782;314.159265358979 314.159265358979 314.159265358979;1.08311699054254 -0.106589276188758 -1.67747481070777]  x4=[0.0547952312750418 537.545390970789 537.599143150521;314.159265358979 314.159265358979 314.159265358979;1.45920867346669 -0.111674569190641 -1.68244934608198]  x5=5.08443513939426e-06  V1=ones(3,3)  V2=ones(3,3)  I1=ones(3,3)  I2=ones(3,3)  nHarmo=1  Measurements=None  Decoupling=off  VsMag0=0  VrMag0=0  VsAngle0=0  VrAngle0=0  IsMag0=0  IrMag0=0  IsAngle0=0  IrAngle0=0
      settings: SourceProductBaseCode=PS
  Line 13 : spsDistributedParametersLineLib/Distributed Parameters Line  Phases=3  Length=0.34002  Frequency=50  Resistance=[0.646656091154803 0.0486237908083191 0.0486712220507153;0.0486237908083191 0.646561225344642 0.0486237934466192;0.0486712220507153 0.0486237934466192 0.646656091154803]  Inductance=[0.00282448912315926 0.00133270803418135 0.00132951476746136;0.00133270803418135 0.00282479813276775 0.00133799988507366;0.00132951476746136 0.00133799988507366 0.00282448912315926]  Capacitance=[7.89543174552926e-09 -1.85986777702161e-09 -1.7901190036642e-09;-1.85986777702161e-09 7.82540023894543e-09 -1.8957321828871e-09;-1.7901190036642e-09 -1.8957321828871e-09 7.91264394645417e-09]  x1=[131.786253662837 9842.40708440789 9841.92739858518;314.159265358979 314.159265358979 314.159265358979;1.06966431092015 2.25877893998269 -2.45335935506964]  x2=[131.787551642506 9842.15744190595 9841.6783147578;314.159265358979 314.159265358979 314.159265358979;1.06967470495036 2.2587755667215 -2.45336263834382]  x3=[0.117989904242175 24.204864523567 24.3958550737452;314.159265358979 314.159265358979 314.159265358979;1.06078144227001 2.27904322656008 -2.43325420274688]  x4=[0.112432759018824 25.8805723739286 26.071513192924;314.159265358979 314.159265358979 314.159265358979;1.07847238501307 2.2394301227809 -2.47256930423816]  x5=1.62919655174204e-06  V1=ones(3,3)  V2=ones(3,3)  I1=ones(3,3)  I2=ones(3,3)  nHarmo=1  Measurements=None  Decoupling=off  VsMag0=0  VrMag0=0  VsAngle0=0  VrAngle0=0  IsMag0=0  IrMag0=0  IsAngle0=0  IrAngle0=0
      settings: SourceProductBaseCode=PS
  Line 130 : spsDistributedParametersLineLib/Distributed Parameters Line  Phases=3  Length=0.02  Frequency=50  Resistance=[0.476003738225748 0.351747138225748 0.351747138225748;0.351747138225748 0.476003738225748 0.351747138225748;0.351747138225748 0.351747138225748 0.476003738225748]  Inductance=[0.000705954362986426 0.000459934243504405 0.000459934243504405;0.000459934243504405 0.000705954362986426 0.000459934243504405;0.000459934243504405 0.000459934243504405 0.000705954362986426]  Capacitance=[5.7561313269996e-07 -1.37543883484145e-07 -1.37543912800485e-07;-1.37543883484145e-07 5.75613027339387e-07 -1.37543875208088e-07;-1.37543912800485e-07 -1.37543875208088e-07 5.75613005057695e-07]  x1=[3.80333987230669 9843.27748434497 9843.52712634007;314.159265358979 314.159265358979 314.159265358979;1.32176499350784 2.17733521648347 -2.53495637814892]  x2=[3.80334430622167 9843.2740131217 9843.523656068;314.159265358979 314.159265358979 314.159265358979;1.32176089945518 2.17733495297998 -2.53495664176215]  x3=[0.0516183148501051 528.436472599349 528.449940379562;314.159265358979 314.159265358979 314.159265358979;1.30960098696501 2.17705489432954 -2.53523764818223]  x4=[0.0517830954145226 531.38652924776 531.399858722047;314.159265358979 314.159265358979 314.159265358979;1.33374752643121 2.17753072210706 -2.53475992991396]  x5=4.42086352438419e-07  V1=ones(3,3)  V2=ones(3,3)  I1=ones(3,3)  I2=ones(3,3)  nHarmo=1  Measurements=None  Decoupling=off  VsMag0=0  VrMag0=0  VsAngle0=0  VrAngle0=0  IsMag0=0  IrMag0=0  IsAngle0=0  IrAngle0=0
      settings: SourceProductBaseCode=PS
  Line 131 : spsDistributedParametersLineLib/Distributed Parameters Line  Phases=3  Length=0.23  Frequency=50  Resistance=[0.646656091154803 0.0486237908083191 0.0486712220507153;0.0486237908083191 0.646561225344642 0.0486237934466192;0.0486712220507153 0.0486237934466192 0.646656091154803]  Inductance=[0.00282448912315926 0.00133270803418135 0.00132951476746136;0.00133270803418135 0.00282479813276775 0.00133799988507366;0.00132951476746136 0.00133799988507366 0.00282448912315926]  Capacitance=[7.89543174552926e-09 -1.85986777702161e-09 -1.7901190036642e-09;-1.85986777702161e-09 7.82540023894543e-09 -1.8957321828871e-09;-1.7901190036642e-09 -1.8957321828871e-09 7.91264394645417e-09]  x1=[132.144359633141 9828.68721827299 9828.83158364109;314.159265358979 314.159265358979 314.159265358979;1.01385121648998 -0.191365391664741 -1.76234303517515]  x2=[132.163450439569 9828.04961373003 9828.20063661273;314.159265358979 314.159265358979 314.159265358979;1.01381255886069 -0.191411476795203 -1.76238953453853]  x3=[0.130325197025453 20.5417070109271 20.7367271561117;314.159265358979 314.159265358979 314.159265358979;0.658359591242439 -0.180982111811502 -1.75473588655404]  x4=[0.117943778758405 29.471341189591 29.6602183170572;314.159265358979 314.159265358979 314.159265358979;1.40820510610179 -0.198875031477451 -1.76793490740146]  x5=1.10203872390056e-06  V1=ones(3,3)  V2=ones(3,3)  I1=ones(3,3)  I2=ones(3,3)  nHarmo=1  Measurements=None  Decoupling=off  VsMag0=0  VrMag0=0  VsAngle0=0  VrAngle0=0  IsMag0=0  IrMag0=0  IsAngle0=0  IrAngle0=0
      settings: SourceProductBaseCode=PS
  Line 132 : spsDistributedParametersLineLib/Distributed Parameters Line  Phases=3  Length=1.62  Frequency=50  Resistance=[0.80718830189013 0.0486237908083191 0.0486712220507153;0.0486237908083191 0.807093436079969 0.0486237934466192;0.0486712220507153 0.0486237934466192 0.80718830189013]  Inductance=[0.00279786707424938 0.00133270803418135 0.00132951476746136;0.00133270803418135 0.00279817608385787 0.00133799988507366;0.00132951476746136 0.00133799988507366 0.00279786707424938]  Capacitance=[7.73340098830622e-09 -1.79942827973291e-09 -1.73218055098733e-09;-1.79942827973291e-09 7.66505189233746e-09 -1.83375898618858e-09;-1.73218055098733e-09 -1.83375898618858e-09 7.749673531177e-09]  x1=[55.4862020307275 9828.7718707264 9828.99604819689;314.159265358979 314.159265358979 314.159265358979;1.07753607946283 -0.197300357750235 -1.76823949589757]  x2=[55.4866732784249 9828.76537719545 9828.98963146268;314.159265358979 314.159265358979 314.159265358979;1.07753587910984 -0.19730313079807 -1.76824228725039]  x3=[0.0483752661832953 24.8778549567773 25.0677176141269;314.159265358979 314.159265358979 314.159265358979;1.07354936951872 -0.198806142312202 -1.76974992058364]  x4=[0.0482417673218573 24.9051881104345 25.095060069947;314.159265358979 314.159265358979 314.159265358979;1.07910908444547 -0.197697484661193 -1.7686336167053]  x5=7.70442045759223e-06  V1=ones(3,3)  V2=ones(3,3)  I1=ones(3,3)  I2=ones(3,3)  nHarmo=1  Measurements=None  Decoupling=off  VsMag0=0  VrMag0=0  VsAngle0=0  VrAngle0=0  IsMag0=0  IrMag0=0  IsAngle0=0  IrAngle0=0
      settings: SourceProductBaseCode=PS
  Line 133 : spsDistributedParametersLineLib/Distributed Parameters Line  Phases=3  Length=0.54002  Frequency=50  Resistance=[0.646656091154803 0.0486237908083191 0.0486712220507153;0.0486237908083191 0.646561225344642 0.0486237934466192;0.0486712220507153 0.0486237934466192 0.646656091154803]  Inductance=[0.00282448912315926 0.00133270803418135 0.00132951476746136;0.00133270803418135 0.00282479813276775 0.00133799988507366;0.00132951476746136 0.00133799988507366 0.00282448912315926]  Capacitance=[7.89543174552926e-09 -1.85986777702161e-09 -1.7901190036642e-09;-1.85986777702161e-09 7.82540023894543e-09 -1.8957321828871e-09;-1.7901190036642e-09 -1.8957321828871e-09 7.91264394645417e-09]  x1=[132.099178478359 9830.17632578495 9830.30501827977;314.159265358979 314.159265358979 314.159265358979;1.01347625666342 -0.191625984363414 -1.76260299427252]  x2=[132.144359633141 9828.68721827299 9828.8315836411;314.159265358979 314.159265358979 314.159265358979;1.01338454786458 -0.191736129237754 -1.76271412566408]  x3=[0.130435444200504 20.5235336816912 20.7185496668985;314.159265358979 314.159265358979 314.159265358979;0.655071041559845 -0.183826140769875 -1.75758267532267]  x4=[0.118015851190294 29.4764634797477 29.6652826879634;314.159265358979 314.159265358979 314.159265358979;1.41064710869762 -0.197697971158661 -1.7667526336238]  x5=2.58749109426427e-06  V1=ones(3,3)  V2=ones(3,3)  I1=ones(3,3)  I2=ones(3,3)  nHarmo=1  Measurements=None  Decoupling=off  VsMag0=0  VrMag0=0  VsAngle0=0  VrAngle0=0  IsMag0=0  IrMag0=0  IsAngle0=0  IrAngle0=0
      settings: SourceProductBaseCode=PS
  Line 134 : spsDistributedParametersLineLib/Distributed Parameters Line  Phases=3  Length=0.13998  Frequency=50  Resistance=[0.646656091154803 0.0486237908083191 0.0486712220507153;0.0486237908083191 0.646561225344642 0.0486237934466192;0.0486712220507153 0.0486237934466192 0.646656091154803]  Inductance=[0.00282448912315926 0.00133270803418135 0.00132951476746136;0.00133270803418135 0.00282479813276775 0.00133799988507366;0.00132951476746136 0.00133799988507366 0.00282448912315926]  Capacitance=[7.89543174552926e-09 -1.85986777702161e-09 -1.7901190036642e-09;-1.85986777702161e-09 7.82540023894543e-09 -1.8957321828871e-09;-1.7901190036642e-09 -1.8957321828871e-09 7.91264394645417e-09]  x1=[132.099178478359 9830.17632578495 9830.30501827977;314.159265358979 314.159265358979 314.159265358979;1.0140784310938 -0.1911475963281 -1.76212415084568]  x2=[132.100593876995 9829.96119389448 9830.09017626153;314.159265358979 314.159265358979 314.159265358979;1.0140852323939 -0.191156006046792 -1.76213247711881]  x3=[0.120823837823496 22.9528402773031 23.1445458384395;314.159265358979 314.159265358979 314.159265358979;0.984207967268187 -0.163428185955141 -1.73465557163936]  x4=[0.110271705994474 27.0884523510253 27.2814160044662;314.159265358979 314.159265358979 314.159265358979;1.04659455942319 -0.214796602157904 -1.78558920357609]  x5=6.70710350311308e-07  V1=ones(3,3)  V2=ones(3,3)  I1=ones(3,3)  I2=ones(3,3)  nHarmo=1  Measurements=None  Decoupling=off  VsMag0=0  VrMag0=0  VsAngle0=0  VrAngle0=0  IsMag0=0  IrMag0=0  IsAngle0=0  IrAngle0=0
      settings: SourceProductBaseCode=PS
  Line 135 : spsDistributedParametersLineLib/Distributed Parameters Line  Phases=3  Length=0.14997  Frequency=50  Resistance=[0.476003738225748 0.351747138225748 0.351747138225748;0.351747138225748 0.476003738225748 0.351747138225748;0.351747138225748 0.351747138225748 0.476003738225748]  Inductance=[0.000705954362986426 0.000459934243504405 0.000459934243504405;0.000459934243504405 0.000705954362986426 0.000459934243504405;0.000459934243504405 0.000459934243504405 0.000705954362986426]  Capacitance=[5.7561313269996e-07 -1.37543883484145e-07 -1.37543912800485e-07;-1.37543883484145e-07 5.75613027339387e-07 -1.37543875208088e-07;-1.37543912800485e-07 -1.37543875208088e-07 5.75613005057695e-07]  x1=[4.31449173622565 9831.0100696163 9831.97047263499;314.159265358979 314.159265358979 314.159265358979;1.28304801672937 -0.109959891680753 -1.68079335624655]  x2=[4.31449407811757 9830.96218524263 9831.92258358313;314.159265358979 314.159265358979 314.159265358979;1.28304676690648 -0.109960804640553 -1.6807942692063]  x3=[0.0585532145619265 526.838788087674 526.890214731611;314.159265358979 314.159265358979 314.159265358979;1.28200674787984 -0.108745672724538 -1.67957913709891]  x4=[0.0585531499615314 530.972220424401 531.024050869575;314.159265358979 314.159265358979 314.159265358979;1.28304597790055 -0.111787362951304 -1.68262082765788]  x5=3.31498451375949e-06  V1=ones(3,3)  V2=ones(3,3)  I1=ones(3,3)  I2=ones(3,3)  nHarmo=1  Measurements=None  Decoupling=off  VsMag0=0  VrMag0=0  VsAngle0=0  VrAngle0=0  IsMag0=0  IrMag0=0  IsAngle0=0  IrAngle0=0
      settings: SourceProductBaseCode=PS
  Line 136 : spsDistributedParametersLineLib/Distributed Parameters Line  Phases=3  Length=1.7101  Frequency=50  Resistance=[0.646656091154803 0.0486237908083191 0.0486712220507153;0.0486237908083191 0.646561225344642 0.0486237934466192;0.0486712220507153 0.0486237934466192 0.646656091154803]  Inductance=[0.00282448912315926 0.00133270803418135 0.00132951476746136;0.00133270803418135 0.00282479813276775 0.00133799988507366;0.00132951476746136 0.00133799988507366 0.00282448912315926]  Capacitance=[7.89543174552926e-09 -1.85986777702161e-09 -1.7901190036642e-09;-1.85986777702161e-09 7.82540023894543e-09 -1.8957321828871e-09;-1.7901190036642e-09 -1.8957321828871e-09 7.91264394645417e-09]  x1=[131.780254208923 9843.54629581266 9843.0641121035;314.159265358979 314.159265358979 314.159265358979;1.06755377729245 2.25715945891224 -2.45498080679507]  x2=[131.783099780823 9842.17764247951 9841.69480280184;314.159265358979 314.159265358979 314.159265358979;1.06765347401386 2.25702095060697 -2.45511856856697]  x3=[0.119237826915875 23.5293347361977 23.7195260537135;314.159265358979 314.159265358979 314.159265358979;1.07308263427041 2.2486962380213 -2.46339920560131]  x4=[0.111018904449141 26.4722480432539 26.6628761177784;314.159265358979 314.159265358979 314.159265358979;1.05904877359913 2.26261840507624 -2.44955714138019]  x5=8.19389748583632e-06  V1=ones(3,3)  V2=ones(3,3)  I1=ones(3,3)  I2=ones(3,3)  nHarmo=1  Measurements=None  Decoupling=off  VsMag0=0  VrMag0=0  VsAngle0=0  VrAngle0=0  IsMag0=0  IrMag0=0  IsAngle0=0  IrAngle0=0
      settings: SourceProductBaseCode=PS
  Line 137 : spsDistributedParametersLineLib/Distributed Parameters Line  Phases=3  Length=0.50001  Frequency=50  Resistance=[0.646656091154803 0.0486237908083191 0.0486712220507153;0.0486237908083191 0.646561225344642 0.0486237934466192;0.0486712220507153 0.0486237934466192 0.646656091154803]  Inductance=[0.00282448912315926 0.00133270803418135 0.00132951476746136;0.00133270803418135 0.00282479813276775 0.00133799988507366;0.00132951476746136 0.00133799988507366 0.00282448912315926]  Capacitance=[7.89543174552926e-09 -1.85986777702161e-09 -1.7901190036642e-09;-1.85986777702161e-09 7.82540023894543e-09 -1.8957321828871e-09;-1.7901190036642e-09 -1.8957321828871e-09 7.91264394645417e-09]  x1=[132.052201438456 9832.31955445955 9832.43269368207;314.159265358979 314.159265358979 314.159265358979;1.01359744166871 -0.191445622758308 -1.76242196711282]  x2=[132.099178478359 9830.17632578495 9830.30501827977;314.159265358979 314.159265358979 314.159265358979;1.01353648313817 -0.19157813838478 -1.76255510274791]  x3=[0.136645487205426 18.4778895635962 18.6702043238108;314.159265358979 314.159265358979 314.159265358979;0.64330292108119 -0.149113197617188 -1.72356438314749]  x4=[0.114681348650533 31.5591626672169 31.7474645243538;314.159265358979 314.159265358979 314.159265358979;1.45851248142746 -0.216805409615927 -1.78585069002866]  x5=2.3957842710327e-06  V1=ones(3,3)  V2=ones(3,3)  I1=ones(3,3)  I2=ones(3,3)  nHarmo=1  Measurements=None  Decoupling=off  VsMag0=0  VrMag0=0  VsAngle0=0  VrAngle0=0  IsMag0=0  IrMag0=0  IsAngle0=0  IrAngle0=0
      settings: SourceProductBaseCode=PS
  Line 138 : spsDistributedParametersLineLib/Distributed Parameters Line  Phases=3  Length=0.17  Frequency=50  Resistance=[0.646656091154803 0.0486237908083191 0.0486712220507153;0.0486237908083191 0.646561225344642 0.0486237934466192;0.0486712220507153 0.0486237934466192 0.646656091154803]  Inductance=[0.00282448912315926 0.00133270803418135 0.00132951476746136;0.00133270803418135 0.00282479813276775 0.00133799988507366;0.00132951476746136 0.00133799988507366 0.00282448912315926]  Capacitance=[7.89543174552926e-09 -1.85986777702161e-09 -1.7901190036642e-09;-1.85986777702161e-09 7.82540023894543e-09 -1.8957321828871e-09;-1.7901190036642e-09 -1.8957321828871e-09 7.91264394645417e-09]  x1=[132.052201438456 9832.31955445955 9832.43269368207;314.159265358979 314.159265358979 314.159265358979;1.0140942009522 -0.191050980133736 -1.76202694881642]  x2=[132.053275242252 9832.14845042591 9832.26173988092;314.159265358979 314.159265358979 314.159265358979;1.01410112672432 -0.19106054589197 -1.76203644125167]  x3=[0.119433279306795 23.5285475378006 23.72055047692;314.159265358979 314.159265358979 314.159265358979;0.997582573566648 -0.180709182459992 -1.75178643199469]  x4=[0.111497476298838 26.5080822309193 26.7008513058224;314.159265358979 314.159265358979 314.159265358979;1.03152331446885 -0.200431223524002 -1.77132550979111]  x5=8.14550361143895e-07  V1=ones(3,3)  V2=ones(3,3)  I1=ones(3,3)  I2=ones(3,3)  nHarmo=1  Measurements=None  Decoupling=off  VsMag0=0  VrMag0=0  VsAngle0=0  VrAngle0=0  IsMag0=0  IrMag0=0  IsAngle0=0  IrAngle0=0
      settings: SourceProductBaseCode=PS
  Line 139 : spsDistributedParametersLineLib/Distributed Parameters Line  Phases=3  Length=0.27999  Frequency=50  Resistance=[0.646656091154803 0.0486237908083191 0.0486712220507153;0.0486237908083191 0.646561225344642 0.0486237934466192;0.0486712220507153 0.0486237934466192 0.646656091154803]  Inductance=[0.00282448912315926 0.00133270803418135 0.00132951476746136;0.00133270803418135 0.00282479813276775 0.00133799988507366;0.00132951476746136 0.00133799988507366 0.00282448912315926]  Capacitance=[7.89543174552926e-09 -1.85986777702161e-09 -1.7901190036642e-09;-1.85986777702161e-09 7.82540023894543e-09 -1.8957321828871e-09;-1.7901190036642e-09 -1.8957321828871e-09 7.91264394645417e-09]  x1=[132.024087588405 9833.79972311697 9833.90390262215;314.159265358979 314.159265358979 314.159265358979;1.01395150961137 -0.191092340355798 -1.76206820568441]  x2=[132.052201438456 9832.31955445955 9832.43269368207;314.159265358979 314.159265358979 314.159265358979;1.01392863459484 -0.191182511730586 -1.76215860562203]  x3=[0.14106672706257 17.0109438348748 17.2017936585978;314.159265358979 314.159265358979 314.159265358979;0.640427539474924 -0.131226763849435 -1.70619718741625]  x4=[0.112020574548127 33.0676515184735 33.2560732631824;314.159265358979 314.159265358979 314.159265358979;1.49088436439994 -0.222197062654463 -1.79127935102519]  x5=1.341564444804e-06  V1=ones(3,3)  V2=ones(3,3)  I1=ones(3,3)  I2=ones(3,3)  nHarmo=1  Measurements=None  Decoupling=off  VsMag0=0  VrMag0=0  VsAngle0=0  VrAngle0=0  IsMag0=0  IrMag0=0  IsAngle0=0  IrAngle0=0
      settings: SourceProductBaseCode=PS
  Line 14 : spsDistributedParametersLineLib/Distributed Parameters Line  Phases=3  Length=0.12001  Frequency=50  Resistance=[0.646656091154803 0.0486237908083191 0.0486712220507153;0.0486237908083191 0.646561225344642 0.0486237934466192;0.0486712220507153 0.0486237934466192 0.646656091154803]  Inductance=[0.00282448912315926 0.00133270803418135 0.00132951476746136;0.00133270803418135 0.00282479813276775 0.00133799988507366;0.00132951476746136 0.00133799988507366 0.00282448912315926]  Capacitance=[7.89543174552926e-09 -1.85986777702161e-09 -1.7901190036642e-09;-1.85986777702161e-09 7.82540023894543e-09 -1.8957321828871e-09;-1.7901190036642e-09 -1.8957321828871e-09 7.91264394645417e-09]  x1=[131.787551642506 9842.15744190595 9841.6783147578;314.159265358979 314.159265358979 314.159265358979;1.07000588282363 2.25903866579072 -2.45309928882292]  x2=[131.787695383983 9842.12544509725 9841.64638200521;314.159265358979 314.159265358979 314.159265358979;1.07000729035614 2.25903816017623 -2.45309978210732]  x3=[0.116229986245485 24.73504832312 24.926143919944;314.159265358979 314.159265358979 314.159265358979;1.06767820879528 2.26599147407393 -2.4461964249662]  x4=[0.114210190986697 25.3536369267386 25.5447251880785;314.159265358979 314.159265358979 314.159265358979;1.07219389133552 2.25211322855982 -2.45997739811353]  x5=5.75024640240464e-07  V1=ones(3,3)  V2=ones(3,3)  I1=ones(3,3)  I2=ones(3,3)  nHarmo=1  Measurements=None  Decoupling=off  VsMag0=0  VrMag0=0  VsAngle0=0  VrAngle0=0  IsMag0=0  IrMag0=0  IsAngle0=0  IrAngle0=0
      settings: SourceProductBaseCode=PS
  Line 140 : spsDistributedParametersLineLib/Distributed Parameters Line  Phases=3  Length=0.28003  Frequency=50  Resistance=[0.476003738225748 0.351747138225748 0.351747138225748;0.351747138225748 0.476003738225748 0.351747138225748;0.351747138225748 0.351747138225748 0.476003738225748]  Inductance=[0.000705954362986426 0.000459934243504405 0.000459934243504405;0.000459934243504405 0.000705954362986426 0.000459934243504405;0.000459934243504405 0.000459934243504405 0.000705954362986426]  Capacitance=[5.7561313269996e-07 -1.37543883484145e-07 -1.37543912800485e-07;-1.37543883484145e-07 5.75613027339387e-07 -1.37543875208088e-07;-1.37543912800485e-07 -1.37543875208088e-07 5.75613005057695e-07]  x1=[4.54470074903476 9824.69388809356 9825.69440909867;314.159265358979 314.159265358979 314.159265358979;1.27858516573108 -0.111013424836071 -1.68184933676476]  x2=[4.54471299969198 9824.70109840143 9825.70162310895;314.159265358979 314.159265358979 314.159265358979;1.27856385357303 -0.111014604536241 -1.68185051728918]  x3=[0.0615063015173295 528.221978778896 528.275688141883;314.159265358979 314.159265358979 314.159265358979;1.27338531662315 -0.11222636990047 -1.68306267166638]  x4=[0.0616570232348241 528.22193615564 528.275731120304;314.159265358979 314.159265358979 314.159265358979;1.28180660713369 -0.110967490625358 -1.68180301355272]  x5=6.18987206366653e-06  V1=ones(3,3)  V2=ones(3,3)  I1=ones(3,3)  I2=ones(3,3)  nHarmo=1  Measurements=None  Decoupling=off  VsMag0=0  VrMag0=0  VsAngle0=0  VrAngle0=0  IsMag0=0  IrMag0=0  IsAngle0=0  IrAngle0=0
      settings: SourceProductBaseCode=PS
  Line 141 : spsDistributedParametersLineLib/Distributed Parameters Line  Phases=3  Length=0.28003  Frequency=50  Resistance=[0.646656091154803 0.0486237908083191 0.0486712220507153;0.0486237908083191 0.646561225344642 0.0486237934466192;0.0486712220507153 0.0486237934466192 0.646656091154803]  Inductance=[0.00282448912315926 0.00133270803418135 0.00132951476746136;0.00133270803418135 0.00282479813276775 0.00133799988507366;0.00132951476746136 0.00133799988507366 0.00282448912315926]  Capacitance=[7.89543174552926e-09 -1.85986777702161e-09 -1.7901190036642e-09;-1.85986777702161e-09 7.82540023894543e-09 -1.8957321828871e-09;-1.7901190036642e-09 -1.8957321828871e-09 7.91264394645417e-09]  x1=[132.244397875019 9823.6512758896 9823.82474595636;314.159265358979 314.159265358979 314.159265358979;1.01372811099302 -0.191837292174622 -1.76281571393209]  x2=[132.244455250325 9823.65400287869 9823.8274780336;314.159265358979 314.159265358979 314.159265358979;1.01372792562905 -0.191837645368685 -1.76281607007926]  x3=[0.115610628180785 24.9921389577793 25.1844776059957;314.159265358979 314.159265358979 314.159265358979;1.01248953781425 -0.192833797561583 -1.76381310000647]  x4=[0.115609824602562 24.9921393996439 25.1844771911872;314.159265358979 314.159265358979 314.159265358979;1.01454496170157 -0.191176049682901 -1.7621539127546]  x5=1.3417561037125e-06  V1=ones(3,3)  V2=ones(3,3)  I1=ones(3,3)  I2=ones(3,3)  nHarmo=1  Measurements=None  Decoupling=off  VsMag0=0  VrMag0=0  VsAngle0=0  VrAngle0=0  IsMag0=0  IrMag0=0  IsAngle0=0  IrAngle0=0
      settings: SourceProductBaseCode=PS
  Line 142 : spsDistributedParametersLineLib/Distributed Parameters Line  Phases=3  Length=0.3  Frequency=50  Resistance=[0.80718830189013 0.0486237908083191 0.0486712220507153;0.0486237908083191 0.807093436079969 0.0486237934466192;0.0486712220507153 0.0486237934466192 0.80718830189013]  Inductance=[0.00279786707424938 0.00133270803418135 0.00132951476746136;0.00133270803418135 0.00279817608385787 0.00133799988507366;0.00132951476746136 0.00133799988507366 0.00279786707424938]  Capacitance=[7.73340098830622e-09 -1.79942827973291e-09 -1.73218055098733e-09;-1.79942827973291e-09 7.66505189233746e-09 -1.83375898618858e-09;-1.73218055098733e-09 -1.83375898618858e-09 7.749673531177e-09]  x1=[55.6282110815718 9823.7385990168 9823.99238724807;314.159265358979 314.159265358979 314.159265358979;1.07976221186629 -0.196166215187824 -1.7671047710465]  x2=[55.6282166695766 9823.73920585724 9823.99299513007;314.159265358979 314.159265358979 314.159265358979;1.07976215894549 -0.196166316686366 -1.76710487339029]  x3=[0.0484694846725867 24.9262226562623 25.1167882634192;314.159265358979 314.159265358979 314.159265358979;1.07931396057819 -0.19651775665592 -1.76745660990567]  x4=[0.0484694846843416 24.9262226565854 25.1167882636431;314.159265358979 314.159265358979 314.159265358979;1.07976215877964 -0.196166316684709 -1.76710487338848]  x5=1.42674452918375e-06  V1=ones(3,3)  V2=ones(3,3)  I1=ones(3,3)  I2=ones(3,3)  nHarmo=1  Measurements=None  Decoupling=off  VsMag0=0  VrMag0=0  VsAngle0=0  VrAngle0=0  IsMag0=0  IrMag0=0  IsAngle0=0  IrAngle0=0
      settings: SourceProductBaseCode=PS
  Line 143 : spsDistributedParametersLineLib/Distributed Parameters Line  Phases=3  Length=0.26  Frequency=50  Resistance=[0.646656091154803 0.0486237908083191 0.0486712220507153;0.0486237908083191 0.646561225344642 0.0486237934466192;0.0486712220507153 0.0486237934466192 0.646656091154803]  Inductance=[0.00282448912315926 0.00133270803418135 0.00132951476746136;0.00133270803418135 0.00282479813276775 0.00133799988507366;0.00132951476746136 0.00133799988507366 0.00282448912315926]  Capacitance=[7.89543174552926e-09 -1.85986777702161e-09 -1.7901190036642e-09;-1.85986777702161e-09 7.82540023894543e-09 -1.8957321828871e-09;-1.7901190036642e-09 -1.8957321828871e-09 7.91264394645417e-09]  x1=[132.244455250325 9823.65400287869 9823.8274780336;314.159265358979 314.159265358979 314.159265358979;1.01375807649856 -0.191813692483105 -1.76279209439222]  x2=[132.244465378525 9823.65447771458 9823.82795378235;314.159265358979 314.159265358979 314.159265358979;1.01375804347038 -0.191813753981523 -1.76279215641097]  x3=[0.115611324109492 24.9927061433613 25.1850530377017;314.159265358979 314.159265358979 314.159265358979;1.01336668562434 -0.192124644361699 -1.76310334250803]  x4=[0.115611324121744 24.9927061434585 25.1850530378551;314.159265358979 314.159265358979 314.159265358979;1.01375804358901 -0.191813753983471 -1.76279215641012]  x5=1.2457829052789e-06  V1=ones(3,3)  V2=ones(3,3)  I1=ones(3,3)  I2=ones(3,3)  nHarmo=1  Measurements=None  Decoupling=off  VsMag0=0  VrMag0=0  VsAngle0=0  VrAngle0=0  IsMag0=0  IrMag0=0  IsAngle0=0  IrAngle0=0
      settings: SourceProductBaseCode=PS
  Line 144 : spsDistributedParametersLineLib/Distributed Parameters Line  Phases=3  Length=0.02  Frequency=50  Resistance=[0.476003738225748 0.351747138225748 0.351747138225748;0.351747138225748 0.476003738225748 0.351747138225748;0.351747138225748 0.351747138225748 0.476003738225748]  Inductance=[0.000705954362986426 0.000459934243504405 0.000459934243504405;0.000459934243504405 0.000705954362986426 0.000459934243504405;0.000459934243504405 0.000459934243504405 0.000705954362986426]  Capacitance=[5.7561313269996e-07 -1.37543883484145e-07 -1.37543912800485e-07;-1.37543883484145e-07 5.75613027339387e-07 -1.37543875208088e-07;-1.37543912800485e-07 -1.37543875208088e-07 5.75613005057695e-07]  x1=[4.54469874191592 9824.69548978742 9825.69601044679;314.159265358979 314.159265358979 314.159265358979;1.28039451630579 -0.109931193188946 -1.68076710505805]  x2=[4.54470074903476 9824.69388809356 9825.69440909867;314.159265358979 314.159265358979 314.159265358979;1.28039088586756 -0.10993136515216 -1.6807672771645]  x3=[0.0615936208803784 528.141704238392 528.19534175087;314.159265358979 314.159265358979 314.159265358979;1.27026034406473 -0.110353660622416 -1.68119051947548]  x4=[0.0619602838959773 529.680726138589 529.734733058749;314.159265358979 314.159265358979 314.159265358979;1.29032660857963 -0.109593232604993 -1.68042820053044]  x5=4.42086352438419e-07  V1=ones(3,3)  V2=ones(3,3)  I1=ones(3,3)  I2=ones(3,3)  nHarmo=1  Measurements=None  Decoupling=off  VsMag0=0  VrMag0=0  VsAngle0=0  VrAngle0=0  IsMag0=0  IrMag0=0  IsAngle0=0  IrAngle0=0
      settings: SourceProductBaseCode=PS
  Line 145 : spsDistributedParametersLineLib/Distributed Parameters Line  Phases=3  Length=1.7101  Frequency=50  Resistance=[0.646656091154803 0.0486237908083191 0.0486712220507153;0.0486237908083191 0.646561225344642 0.0486237934466192;0.0486712220507153 0.0486237934466192 0.646656091154803]  Inductance=[0.00282448912315926 0.00133270803418135 0.00132951476746136;0.00133270803418135 0.00282479813276775 0.00133799988507366;0.00132951476746136 0.00133799988507366 0.00282448912315926]  Capacitance=[7.89543174552926e-09 -1.85986777702161e-09 -1.7901190036642e-09;-1.85986777702161e-09 7.82540023894543e-09 -1.8957321828871e-09;-1.7901190036642e-09 -1.8957321828871e-09 7.91264394645417e-09]  x1=[132.238913203071 9824.23295491704 9824.40694442497;314.159265358979 314.159265358979 314.159265358979;1.01153352005884 -0.193457253790081 -1.76443761592241]  x2=[132.24428286333 9823.6456684323 9823.81913361315;314.159265358979 314.159265358979 314.159265358979;1.01157755770441 -0.193546090405388 -1.76452613918188]  x3=[0.11785860225711 24.1856100115289 24.3772276665275;314.159265358979 314.159265358979 314.159265358979;1.00333035021471 -0.204775972900738 -1.77571704783392]  x4=[0.113201838878256 25.7211067757001 25.9129361755245;314.159265358979 314.159265358979 314.159265358979;1.01749122651595 -0.184885713299888 -1.75590018328428]  x5=8.19389748583632e-06  V1=ones(3,3)  V2=ones(3,3)  I1=ones(3,3)  I2=ones(3,3)  nHarmo=1  Measurements=None  Decoupling=off  VsMag0=0  VrMag0=0  VsAngle0=0  VrAngle0=0  IsMag0=0  IrMag0=0  IsAngle0=0  IrAngle0=0
      settings: SourceProductBaseCode=PS
  Line 146 : spsDistributedParametersLineLib/Distributed Parameters Line  Phases=3  Length=0.02  Frequency=50  Resistance=[0.646656091154803 0.0486237908083191 0.0486712220507153;0.0486237908083191 0.646561225344642 0.0486237934466192;0.0486712220507153 0.0486237934466192 0.646656091154803]  Inductance=[0.00282448912315926 0.00133270803418135 0.00132951476746136;0.00133270803418135 0.00282479813276775 0.00133799988507366;0.00132951476746136 0.00133799988507366 0.00282448912315926]  Capacitance=[7.89543174552926e-09 -1.85986777702161e-09 -1.7901190036642e-09;-1.85986777702161e-09 7.82540023894543e-09 -1.8957321828871e-09;-1.7901190036642e-09 -1.8957321828871e-09 7.91264394645417e-09]  x1=[132.238913203071 9824.23295491704 9824.40694442497;314.159265358979 314.159265358979 314.159265358979;1.01407760316247 -0.191436146854563 -1.7624145850362]  x2=[132.238977295213 9824.22286407437 9824.39686429174;314.159265358979 314.159265358979 314.159265358979;1.01407797519288 -0.191436641168063 -1.76241507518458]  x3=[0.117506247577389 24.2825795695461 24.4748371304669;314.159265358979 314.159265358979 314.159265358979;1.00512750790325 -0.184902324996559 -1.75593926536932]  x4=[0.113743303853166 25.7204538131784 25.9131140735896;314.159265358979 314.159265358979 314.159265358979;1.02329357499585 -0.197628426801093 -1.7685542471849]  x5=9.5829454252223e-08  V1=ones(3,3)  V2=ones(3,3)  I1=ones(3,3)  I2=ones(3,3)  nHarmo=1  Measurements=None  Decoupling=off  VsMag0=0  VrMag0=0  VsAngle0=0  VrAngle0=0  IsMag0=0  IrMag0=0  IsAngle0=0  IrAngle0=0
      settings: SourceProductBaseCode=PS
  Line 147 : spsDistributedParametersLineLib/Distributed Parameters Line  Phases=3  Length=0.02  Frequency=50  Resistance=[0.646656091154803 0.0486237908083191 0.0486712220507153;0.0486237908083191 0.646561225344642 0.0486237934466192;0.0486712220507153 0.0486237934466192 0.646656091154803]  Inductance=[0.00282448912315926 0.00133270803418135 0.00132951476746136;0.00133270803418135 0.00282479813276775 0.00133799988507366;0.00132951476746136 0.00133799988507366 0.00282448912315926]  Capacitance=[7.89543174552926e-09 -1.85986777702161e-09 -1.7901190036642e-09;-1.85986777702161e-09 7.82540023894543e-09 -1.8957321828871e-09;-1.7901190036642e-09 -1.8957321828871e-09 7.91264394645417e-09]  x1=[131.780254208923 9843.54629581266 9843.0641121035;314.159265358979 314.159265358979 314.159265358979;1.07009786039607 2.25918056584775 -2.45295777590887]  x2=[131.780322587806 9843.53223091875 9843.05007950473;314.159265358979 314.159265358979 314.159265358979;1.07009843130723 2.25918047636706 -2.45295786025275]  x3=[0.117786704753444 24.2929843136282 24.4841401002132;314.159265358979 314.159265358979 314.159265358979;1.06261244468216 2.2808196596663 -2.43147573515382]  x4=[0.1126580016633 25.8183768589414 26.0094668584173;314.159265358979 314.159265358979 314.159265358979;1.07789384615804 2.23879683064791 -2.47320314353107]  x5=9.5829454252223e-08  V1=ones(3,3)  V2=ones(3,3)  I1=ones(3,3)  I2=ones(3,3)  nHarmo=1  Measurements=None  Decoupling=off  VsMag0=0  VrMag0=0  VsAngle0=0  VrAngle0=0  IsMag0=0  IrMag0=0  IsAngle0=0  IrAngle0=0
      settings: SourceProductBaseCode=PS
  Line 148 : spsDistributedParametersLineLib/Distributed Parameters Line  Phases=3  Length=0.14997  Frequency=50  Resistance=[0.476003738225748 0.351747138225748 0.351747138225748;0.351747138225748 0.476003738225748 0.351747138225748;0.351747138225748 0.351747138225748 0.476003738225748]  Inductance=[0.000705954362986426 0.000459934243504405 0.000459934243504405;0.000459934243504405 0.000705954362986426 0.000459934243504405;0.000459934243504405 0.000459934243504405 0.000705954362986426]  Capacitance=[5.7561313269996e-07 -1.37543883484145e-07 -1.37543912800485e-07;-1.37543883484145e-07 5.75613027339387e-07 -1.37543875208088e-07;-1.37543912800485e-07 -1.37543875208088e-07 5.75613005057695e-07]  x1=[5.50111428933843 9785.79282545685 9785.90189963939;314.159265358979 314.159265358979 314.159265358979;1.26479806447785 2.17471089169687 -2.53758285426424]  x2=[5.50111726791684 9785.74399966113 9785.85307329915;314.159265358979 314.159265358979 314.159265358979;1.26479681036516 2.17471045484927 -2.5375832911118]  x3=[0.074657128604592 524.483064762699 524.488870074243;314.159265358979 314.159265358979 314.159265358979;1.26375549534279 2.17632177981981 -2.53597196592085]  x4=[0.0746572136308369 528.463246822263 528.469096498785;314.159265358979 314.159265358979 314.159265358979;1.26479731867886 2.17248982681794 -2.5398039193129]  x5=3.31498451375949e-06  V1=ones(3,3)  V2=ones(3,3)  I1=ones(3,3)  I2=ones(3,3)  nHarmo=1  Measurements=None  Decoupling=off  VsMag0=0  VrMag0=0  VsAngle0=0  VrAngle0=0  IsMag0=0  IrMag0=0  IsAngle0=0  IrAngle0=0
      settings: SourceProductBaseCode=PS
  Line 149 : spsDistributedParametersLineLib/Distributed Parameters Line  Phases=3  Length=0.50001  Frequency=50  Resistance=[0.646656091154803 0.0486237908083191 0.0486712220507153;0.0486237908083191 0.646561225344642 0.0486237934466192;0.0486712220507153 0.0486237934466192 0.646656091154803]  Inductance=[0.00282448912315926 0.00133270803418135 0.00132951476746136;0.00133270803418135 0.00282479813276775 0.00133799988507366;0.00132951476746136 0.00133799988507366 0.00282448912315926]  Capacitance=[7.89543174552926e-09 -1.85986777702161e-09 -1.7901190036642e-09;-1.85986777702161e-09 7.82540023894543e-09 -1.8957321828871e-09;-1.7901190036642e-09 -1.8957321828871e-09 7.91264394645417e-09]  x1=[132.717849837094 9787.48797541449 9786.86247601469;314.159265358979 314.159265358979 314.159265358979;1.06824871452495 2.25648753339401 -2.45565068965463]  x2=[132.741273272324 9784.92376829306 9784.30496184118;314.159265358979 314.159265358979 314.159265358979;1.06842967988739 2.25638928564386 -2.45574829246511]  x3=[0.149978933824982 18.1619767428892 18.347627697318;314.159265358979 314.159265358979 314.159265358979;0.982560180756545 2.3763294793653 -2.33777852818396]  x4=[0.0835960752382819 31.8248673386566 32.0138346533611;314.159265358979 314.159265358979 314.159265358979;1.22160048947019 2.18766021272988 -2.52364654504681]  x5=2.3957842710327e-06  V1=ones(3,3)  V2=ones(3,3)  I1=ones(3,3)  I2=ones(3,3)  nHarmo=1  Measurements=None  Decoupling=off  VsMag0=0  VrMag0=0  VsAngle0=0  VrAngle0=0  IsMag0=0  IrMag0=0  IsAngle0=0  IrAngle0=0
      settings: SourceProductBaseCode=PS
  Line 15 : spsDistributedParametersLineLib/Distributed Parameters Line  Phases=3  Length=0.82  Frequency=50  Resistance=[0.646656091154803 0.0486237908083191 0.0486712220507153;0.0486237908083191 0.646561225344642 0.0486237934466192;0.0486712220507153 0.0486237934466192 0.646656091154803]  Inductance=[0.00282448912315926 0.00133270803418135 0.00132951476746136;0.00133270803418135 0.00282479813276775 0.00133799988507366;0.00132951476746136 0.00133799988507366 0.00282448912315926]  Capacitance=[7.89543174552926e-09 -1.85986777702161e-09 -1.7901190036642e-09;-1.85986777702161e-09 7.82540023894543e-09 -1.8957321828871e-09;-1.7901190036642e-09 -1.8957321828871e-09 7.91264394645417e-09]  x1=[131.787551642506 9842.15744190595 9841.6783147578;314.159265358979 314.159265358979 314.159265358979;1.06895219799332 2.25820158239696 -2.45393716906079]  x2=[131.789543045604 9841.76663859446 9841.28840735579;314.159265358979 314.159265358979 314.159265358979;1.06896815946448 2.25819785662097 -2.4539407539794]  x3=[0.116951518879854 24.4972244347383 24.6880229144519;314.159265358979 314.159265358979 314.159265358979;1.06280861547304 2.27161460832502 -2.44062814618719]  x4=[0.113414847888523 25.5539972435541 25.744745737774;314.159265358979 314.159265358979 314.159265358979;1.07404982479102 2.2443790107144 -2.46766507415549]  x5=3.92900762434114e-06  V1=ones(3,3)  V2=ones(3,3)  I1=ones(3,3)  I2=ones(3,3)  nHarmo=1  Measurements=None  Decoupling=off  VsMag0=0  VrMag0=0  VsAngle0=0  VrAngle0=0  IsMag0=0  IrMag0=0  IsAngle0=0  IrAngle0=0
      settings: SourceProductBaseCode=PS
  Line 150 : spsDistributedParametersLineLib/Distributed Parameters Line  Phases=3  Length=0.17  Frequency=50  Resistance=[0.646656091154803 0.0486237908083191 0.0486712220507153;0.0486237908083191 0.646561225344642 0.0486237934466192;0.0486712220507153 0.0486237934466192 0.646656091154803]  Inductance=[0.00282448912315926 0.00133270803418135 0.00132951476746136;0.00133270803418135 0.00282479813276775 0.00133799988507366;0.00132951476746136 0.00133799988507366 0.00282448912315926]  Capacitance=[7.89543174552926e-09 -1.85986777702161e-09 -1.7901190036642e-09;-1.85986777702161e-09 7.82540023894543e-09 -1.8957321828871e-09;-1.7901190036642e-09 -1.8957321828871e-09 7.91264394645417e-09]  x1=[132.717849837094 9787.48797541449 9786.86247601469;314.159265358979 314.159265358979 314.159265358979;1.06874547380844 2.25688217601858 -2.45525567135822]  x2=[132.718274048059 9787.39046243826 9786.76515133001;314.159265358979 314.159265358979 314.159265358979;1.06874982354674 2.25688040430199 -2.45525740462235]  x3=[0.118221449853064 24.2300310677605 24.4196570369842;314.159265358979 314.159265358979 314.159265358979;1.06434936988875 2.27166145162173 -2.4405830388808]  x4=[0.113841624952248 25.5814475168298 25.771048690263;314.159265358979 314.159265358979 314.159265358979;1.07305431495861 2.24268405088839 -2.46935869648952]  x5=8.14550361143895e-07  V1=ones(3,3)  V2=ones(3,3)  I1=ones(3,3)  I2=ones(3,3)  nHarmo=1  Measurements=None  Decoupling=off  VsMag0=0  VrMag0=0  VsAngle0=0  VrAngle0=0  IsMag0=0  IrMag0=0  IsAngle0=0  IrAngle0=0
      settings: SourceProductBaseCode=PS
  Line 151 : spsDistributedParametersLineLib/Distributed Parameters Line  Phases=3  Length=0.27999  Frequency=50  Resistance=[0.646656091154803 0.0486237908083191 0.0486712220507153;0.0486237908083191 0.646561225344642 0.0486237934466192;0.0486712220507153 0.0486237934466192 0.646656091154803]  Inductance=[0.00282448912315926 0.00133270803418135 0.00132951476746136;0.00133270803418135 0.00282479813276775 0.00133799988507366;0.00132951476746136 0.00133799988507366 0.00282448912315926]  Capacitance=[7.89543174552926e-09 -1.85986777702161e-09 -1.7901190036642e-09;-1.85986777702161e-09 7.82540023894543e-09 -1.8957321828871e-09;-1.7901190036642e-09 -1.8957321828871e-09 7.91264394645417e-09]  x1=[132.70399677141 9789.08263689577 9788.45307552198;314.159265358979 314.159265358979 314.159265358979;1.06847150920817 2.25680879617248 -2.45532959861915]  x2=[132.717849837094 9787.48797541449 9786.86247601469;314.159265358979 314.159265358979 314.159265358979;1.06857990745108 2.25675064442173 -2.45538732816384]  x3=[0.152213888625299 17.5473730666129 17.7322334650593;314.159265358979 314.159265358979 314.159265358979;0.980314126536808 2.40102674004923 -2.31339836286661]  x4=[0.0815162863141507 32.5377417169806 32.7265912663069;314.159265358979 314.159265358979 314.159265358979;1.23317106144038 2.17892290646238 -2.53235157482981]  x5=1.341564444804e-06  V1=ones(3,3)  V2=ones(3,3)  I1=ones(3,3)  I2=ones(3,3)  nHarmo=1  Measurements=None  Decoupling=off  VsMag0=0  VrMag0=0  VsAngle0=0  VrAngle0=0  IsMag0=0  IrMag0=0  IsAngle0=0  IrAngle0=0
      settings: SourceProductBaseCode=PS
  Line 152 : spsDistributedParametersLineLib/Distributed Parameters Line  Phases=3  Length=0.28003  Frequency=50  Resistance=[0.476003738225748 0.351747138225748 0.351747138225748;0.351747138225748 0.476003738225748 0.351747138225748;0.351747138225748 0.351747138225748 0.476003738225748]  Inductance=[0.000705954362986426 0.000459934243504405 0.000459934243504405;0.000459934243504405 0.000705954362986426 0.000459934243504405;0.000459934243504405 0.000459934243504405 0.000705954362986426]  Capacitance=[5.7561313269996e-07 -1.37543883484145e-07 -1.37543912800485e-07;-1.37543883484145e-07 5.75613027339387e-07 -1.37543875208088e-07;-1.37543912800485e-07 -1.37543875208088e-07 5.75613005057695e-07]  x1=[5.70282059813818 9777.61614892348 9777.73874302418;314.159265358979 314.159265358979 314.159265358979;1.28090239550408 2.17373534400957 -2.53855591185669]  x2=[5.70285302410737 9777.62332319574 9777.7459233108;314.159265358979 314.159265358979 314.159265358979;1.28088501756289 2.17373416421474 -2.53855709228662]  x3=[0.0772477737126384 525.690814343618 525.697407929995;314.159265358979 314.159265358979 314.159265358979;1.27620275388263 2.17252239878637 -2.53976924666192]  x4=[0.0773010202067162 525.690857184053 525.697365485229;314.159265358979 314.159265358979 314.159265358979;1.28363530952485 2.17378127818244 -2.53850958854445]  x5=6.18987206366653e-06  V1=ones(3,3)  V2=ones(3,3)  I1=ones(3,3)  I2=ones(3,3)  nHarmo=1  Measurements=None  Decoupling=off  VsMag0=0  VrMag0=0  VsAngle0=0  VrAngle0=0  IsMag0=0  IrMag0=0  IsAngle0=0  IrAngle0=0
      settings: SourceProductBaseCode=PS
  Line 153 : spsDistributedParametersLineLib/Distributed Parameters Line  Phases=3  Length=1.11  Frequency=50  Resistance=[0.502970710632245 0.0486237908083191 0.0486712220507153;0.0486237908083191 0.502875844822084 0.0486237934466192;0.0486712220507153 0.0486237934466192 0.502970710632245]  Inductance=[0.00286900545038753 0.00133270803418135 0.00132951476746136;0.00133270803418135 0.00286931445999602 0.00133799988507366;0.00132951476746136 0.00133799988507366 0.00286900545038753]  Capacitance=[8.11484299003193e-09 -1.94249816214699e-09 -1.86930692621136e-09;-1.94249816214699e-09 8.0425699231653e-09 -1.98049571960044e-09;-1.86930692621136e-09 -1.98049571960044e-09 8.13337738722527e-09]  x1=[236.195437631518 9750.98702019459 9751.0536626707;314.159265358979 314.159265358979 314.159265358979;0.991149495123818 -0.189466307517273 -1.76046338606622]  x2=[236.195774394691 9750.99613890071 9751.06280197488;314.159265358979 314.159265358979 314.159265358979;0.99114900291238 -0.189467185319373 -1.76046427142947]  x3=[0.207070862450441 24.8044058056151 24.995031595079;314.159265358979 314.159265358979 314.159265358979;0.989460592616149 -0.190834340509981 -1.76183296190934]  x4=[0.207070862468034 24.8044058129666 24.9950316027082;314.159265358979 314.159265358979 314.159265358979;0.991149002985776 -0.189467185318813 -1.76046427143388]  x5=5.37516004033389e-06  V1=ones(3,3)  V2=ones(3,3)  I1=ones(3,3)  I2=ones(3,3)  nHarmo=1  Measurements=None  Decoupling=off  VsMag0=0  VrMag0=0  VsAngle0=0  VrAngle0=0  IsMag0=0  IrMag0=0  IsAngle0=0  IrAngle0=0
      settings: SourceProductBaseCode=PS
  Line 154 : spsDistributedParametersLineLib/Distributed Parameters Line  Phases=3  Length=0.02  Frequency=50  Resistance=[0.646656091154803 0.0486237908083191 0.0486712220507153;0.0486237908083191 0.646561225344642 0.0486237934466192;0.0486712220507153 0.0486237934466192 0.646656091154803]  Inductance=[0.00282448912315926 0.00133270803418135 0.00132951476746136;0.00133270803418135 0.00282479813276775 0.00133799988507366;0.00132951476746136 0.00133799988507366 0.00282448912315926]  Capacitance=[7.89543174552926e-09 -1.85986777702161e-09 -1.7901190036642e-09;-1.85986777702161e-09 7.82540023894543e-09 -1.8957321828871e-09;-1.7901190036642e-09 -1.8957321828871e-09 7.91264394645417e-09]  x1=[133.233374356816 9752.20427043587 9752.42618752485;314.159265358979 314.159265358979 314.159265358979;1.01368135958762 -0.194154419394454 -1.76512495877769]  x2=[133.233556034884 9752.17913691839 9752.40105493808;314.159265358979 314.159265358979 314.159265358979;1.01368276187795 -0.194156871170561 -1.76512739829396]  x3=[0.123008114409559 22.5479716823281 22.7386852023754;314.159265358979 314.159265358979 314.159265358979;0.993537994594419 -0.203695912581535 -1.77465836858703]  x4=[0.110023750447394 27.0892856545099 27.2809435524574;314.159265358979 314.159265358979 314.159265358979;1.03617191073351 -0.186236680966476 -1.75720307513919]  x5=9.5829454252223e-08  V1=ones(3,3)  V2=ones(3,3)  I1=ones(3,3)  I2=ones(3,3)  nHarmo=1  Measurements=None  Decoupling=off  VsMag0=0  VrMag0=0  VsAngle0=0  VrAngle0=0  IsMag0=0  IrMag0=0  IsAngle0=0  IrAngle0=0
      settings: SourceProductBaseCode=PS
  Line 155 : spsDistributedParametersLineLib/Distributed Parameters Line  Phases=3  Length=1.15  Frequency=50  Resistance=[0.646656091154803 0.0486237908083191 0.0486712220507153;0.0486237908083191 0.646561225344642 0.0486237934466192;0.0486712220507153 0.0486237934466192 0.646656091154803]  Inductance=[0.00282448912315926 0.00133270803418135 0.00132951476746136;0.00133270803418135 0.00282479813276775 0.00133799988507366;0.00132951476746136 0.00133799988507366 0.00282448912315926]  Capacitance=[7.89543174552926e-09 -1.85986777702161e-09 -1.7901190036642e-09;-1.85986777702161e-09 7.82540023894543e-09 -1.8957321828871e-09;-1.7901190036642e-09 -1.8957321828871e-09 7.91264394645417e-09]  x1=[133.233374356816 9752.20427043587 9752.42618752484;314.159265358979 314.159265358979 314.159265358979;1.01198038691908 -0.19550573046311 -1.76647755619879]  x2=[133.243686973268 9750.77438348295 9750.99850922679;314.159265358979 314.159265358979 314.159265358979;1.01202037700812 -0.195560676215336 -1.76653198250194]  x3=[0.120638248932083 23.1286905035743 23.3187868766035;314.159265358979 314.159265358979 314.159265358979;0.982858078888173 -0.173400473307058 -1.74459635158616]  x4=[0.112321663997934 26.4504636233304 26.6416033324668;314.159265358979 314.159265358979 314.159265358979;1.04150557930639 -0.21617542799044 -1.78697157272902]  x5=5.51019361950282e-06  V1=ones(3,3)  V2=ones(3,3)  I1=ones(3,3)  I2=ones(3,3)  nHarmo=1  Measurements=None  Decoupling=off  VsMag0=0  VrMag0=0  VsAngle0=0  VrAngle0=0  IsMag0=0  IrMag0=0  IsAngle0=0  IrAngle0=0
      settings: SourceProductBaseCode=PS
  Line 156 : spsDistributedParametersLineLib/Distributed Parameters Line  Phases=3  Length=0.18999  Frequency=50  Resistance=[0.646656091154803 0.0486237908083191 0.0486712220507153;0.0486237908083191 0.646561225344642 0.0486237934466192;0.0486712220507153 0.0486237934466192 0.646656091154803]  Inductance=[0.00282448912315926 0.00133270803418135 0.00132951476746136;0.00133270803418135 0.00282479813276775 0.00133799988507366;0.00132951476746136 0.00133799988507366 0.00282448912315926]  Capacitance=[7.89543174552926e-09 -1.85986777702161e-09 -1.7901190036642e-09;-1.85986777702161e-09 7.82540023894543e-09 -1.8957321828871e-09;-1.7901190036642e-09 -1.8957321828871e-09 7.91264394645417e-09]  x1=[133.243686973268 9750.77438348295 9750.99850922679;314.159265358979 314.159265358979 314.159265358979;1.01346546618647 -0.194412647773725 -1.76538286121855]  x2=[133.244360018366 9750.67432141735 9750.89861243211;314.159265358979 314.159265358979 314.159265358979;1.01346802283589 -0.194415525661418 -1.76538570281915]  x3=[0.118123086074814 24.1463437617163 24.3371870314948;314.159265358979 314.159265358979 314.159265358979;1.00184296992773 -0.183130302669252 -1.75419627498292]  x4=[0.114870971296148 25.4749991493342 25.6662941974808;314.159265358979 314.159265358979 314.159265358979;1.02512956845551 -0.205330629015924 -1.77621444839129]  x5=9.10331900668992e-07  V1=ones(3,3)  V2=ones(3,3)  I1=ones(3,3)  I2=ones(3,3)  nHarmo=1  Measurements=None  Decoupling=off  VsMag0=0  VrMag0=0  VsAngle0=0  VrAngle0=0  IsMag0=0  IrMag0=0  IsAngle0=0  IrAngle0=0
      settings: SourceProductBaseCode=PS
  Line 157 : spsDistributedParametersLineLib/Distributed Parameters Line  Phases=3  Length=0.34002  Frequency=50  Resistance=[0.646656091154803 0.0486237908083191 0.0486712220507153;0.0486237908083191 0.646561225344642 0.0486237934466192;0.0486712220507153 0.0486237934466192 0.646656091154803]  Inductance=[0.00282448912315926 0.00133270803418135 0.00132951476746136;0.00133270803418135 0.00282479813276775 0.00133799988507366;0.00132951476746136 0.00133799988507366 0.00282448912315926]  Capacitance=[7.89543174552926e-09 -1.85986777702161e-09 -1.7901190036642e-09;-1.85986777702161e-09 7.82540023894543e-09 -1.8957321828871e-09;-1.7901190036642e-09 -1.8957321828871e-09 7.91264394645417e-09]  x1=[133.243686973268 9750.77438348295 9750.99850922679;314.159265358979 314.159265358979 314.159265358979;1.01323962819579 -0.194592061224725 -1.76556244545845]  x2=[133.245445374746 9750.5267098724 9750.75118509633;314.159265358979 314.159265358979 314.159265358979;1.01324715453955 -0.194602639545786 -1.76557293070943]  x3=[0.11903259854133 23.8072217721279 23.9979129994703;314.159265358979 314.159265358979 314.159265358979;0.996945636115581 -0.183117279465298 -1.75420160395783]  x4=[0.113960919038884 25.8053216648957 25.9966283401203;314.159265358979 314.159265358979 314.159265358979;1.02974327691128 -0.205579407185209 -1.77645127628813]  x5=1.62919655174204e-06  V1=ones(3,3)  V2=ones(3,3)  I1=ones(3,3)  I2=ones(3,3)  nHarmo=1  Measurements=None  Decoupling=off  VsMag0=0  VrMag0=0  VsAngle0=0  VrAngle0=0  IsMag0=0  IrMag0=0  IsAngle0=0  IrAngle0=0
      settings: SourceProductBaseCode=PS
  Line 158 : spsDistributedParametersLineLib/Distributed Parameters Line  Phases=3  Length=0.12001  Frequency=50  Resistance=[0.646656091154803 0.0486237908083191 0.0486712220507153;0.0486237908083191 0.646561225344642 0.0486237934466192;0.0486712220507153 0.0486237934466192 0.646656091154803]  Inductance=[0.00282448912315926 0.00133270803418135 0.00132951476746136;0.00133270803418135 0.00282479813276775 0.00133799988507366;0.00132951476746136 0.00133799988507366 0.00282448912315926]  Capacitance=[7.89543174552926e-09 -1.85986777702161e-09 -1.7901190036642e-09;-1.85986777702161e-09 7.82540023894543e-09 -1.8957321828871e-09;-1.7901190036642e-09 -1.8957321828871e-09 7.91264394645417e-09]  x1=[133.245445374746 9750.52670987241 9750.75118509633;314.159265358979 314.159265358979 314.159265358979;1.01357833241283 -0.194339540476569 -1.76530958118853]  x2=[133.245607367443 9750.50140639806 9750.72590542482;314.159265358979 314.159265358979 314.159265358979;1.01357931140279 -0.194340920773019 -1.76531095074463]  x3=[0.117312589814266 24.5015792843339 24.6926035472081;314.159265358979 314.159265358979 314.159265358979;1.0098104424434 -0.192151756146 -1.76314303378634]  x4=[0.115677840248861 25.1197244495933 25.3109175886415;314.159265358979 314.159265358979 314.159265358979;1.01721852683766 -0.196616605816327 -1.76756645784587]  x5=5.75024640240464e-07  V1=ones(3,3)  V2=ones(3,3)  I1=ones(3,3)  I2=ones(3,3)  nHarmo=1  Measurements=None  Decoupling=off  VsMag0=0  VrMag0=0  VsAngle0=0  VrAngle0=0  IsMag0=0  IrMag0=0  IsAngle0=0  IrAngle0=0
      settings: SourceProductBaseCode=PS
  Line 159 : spsDistributedParametersLineLib/Distributed Parameters Line  Phases=3  Length=0.82  Frequency=50  Resistance=[0.646656091154803 0.0486237908083191 0.0486712220507153;0.0486237908083191 0.646561225344642 0.0486237934466192;0.0486712220507153 0.0486237934466192 0.646656091154803]  Inductance=[0.00282448912315926 0.00133270803418135 0.00132951476746136;0.00133270803418135 0.00282479813276775 0.00133799988507366;0.00132951476746136 0.00133799988507366 0.00282448912315926]  Capacitance=[7.89543174552926e-09 -1.85986777702161e-09 -1.7901190036642e-09;-1.85986777702161e-09 7.82540023894543e-09 -1.8957321828871e-09;-1.7901190036642e-09 -1.8957321828871e-09 7.91264394645417e-09]  x1=[133.245445374746 9750.5267098724 9750.75118509633;314.159265358979 314.159265358979 314.159265358979;1.01252464758252 -0.195176623870329 -1.7661474614264]  x2=[133.248420685834 9750.0949918903 9750.32013313421;314.159265358979 314.159265358979 314.159265358979;1.012536621391 -0.19519175001425 -1.76616242841263]  x3=[0.118182226710834 24.1018356259812 24.2924086988723;314.159265358979 314.159265358979 314.159265358979;1.00035994863898 -0.185651299480251 -1.75671137965887]  x4=[0.114745731174966 25.4810550060377 25.6720671118407;314.159265358979 314.159265358979 314.159265358979;1.02381284954655 -0.205155424865008 -1.77604643770912]  x5=3.92900762434114e-06  V1=ones(3,3)  V2=ones(3,3)  I1=ones(3,3)  I2=ones(3,3)  nHarmo=1  Measurements=None  Decoupling=off  VsMag0=0  VrMag0=0  VsAngle0=0  VrAngle0=0  IsMag0=0  IrMag0=0  IsAngle0=0  IrAngle0=0
      settings: SourceProductBaseCode=PS
  Line 16 : spsDistributedParametersLineLib/Distributed Parameters Line  Phases=3  Length=1.11  Frequency=50  Resistance=[0.646656091154803 0.0486237908083191 0.0486712220507153;0.0486237908083191 0.646561225344642 0.0486237934466192;0.0486712220507153 0.0486237934466192 0.646656091154803]  Inductance=[0.00282448912315926 0.00133270803418135 0.00132951476746136;0.00133270803418135 0.00282479813276775 0.00133799988507366;0.00132951476746136 0.00133799988507366 0.00282448912315926]  Capacitance=[7.89543174552926e-09 -1.85986777702161e-09 -1.7901190036642e-09;-1.85986777702161e-09 7.82540023894543e-09 -1.8957321828871e-09;-1.7901190036642e-09 -1.8957321828871e-09 7.91264394645417e-09]  x1=[131.767945414107 9846.34212093538 9845.8560497775;314.159265358979 314.159265358979 314.159265358979;1.06831299430161 2.2579976721775 -2.45414306856435]  x2=[131.78014733242 9843.57612220075 9843.09391339889;314.159265358979 314.159265358979 314.159265358979;1.06845537933645 2.25787882977699 -2.45426076639461]  x3=[0.125758180122261 21.6156229925836 21.8059786021619;314.159265358979 314.159265358979 314.159265358979;1.05313668645833 2.30047889212302 -2.4120689388274]  x4=[0.104575485483517 28.4651286687099 28.6558632309164;314.159265358979 314.159265358979 314.159265358979;1.08488005603969 2.22447023176916 -2.48742960124612]  x5=5.31853471099837e-06  V1=ones(3,3)  V2=ones(3,3)  I1=ones(3,3)  I2=ones(3,3)  nHarmo=1  Measurements=None  Decoupling=off  VsMag0=0  VrMag0=0  VsAngle0=0  VrAngle0=0  IsMag0=0  IrMag0=0  IsAngle0=0  IrAngle0=0
      settings: SourceProductBaseCode=PS
  Line 160 : spsDistributedParametersLineLib/Distributed Parameters Line  Phases=3  Length=1.11  Frequency=50  Resistance=[0.646656091154803 0.0486237908083191 0.0486712220507153;0.0486237908083191 0.646561225344642 0.0486237934466192;0.0486712220507153 0.0486237934466192 0.646656091154803]  Inductance=[0.00282448912315926 0.00133270803418135 0.00132951476746136;0.00133270803418135 0.00282479813276775 0.00133799988507366;0.00132951476746136 0.00133799988507366 0.00282448912315926]  Capacitance=[7.89543174552926e-09 -1.85986777702161e-09 -1.7901190036642e-09;-1.85986777702161e-09 7.82540023894543e-09 -1.8957321828871e-09;-1.7901190036642e-09 -1.8957321828871e-09 7.91264394645417e-09]  x1=[133.212956294541 9754.96187830579 9755.18157544786;314.159265358979 314.159265358979 314.159265358979;1.01192538787568 -0.195266548120737 -1.76623949018326]  x2=[133.233374356816 9752.20427043587 9752.42618752485;314.159265358979 314.159265358979 314.159265358979;1.01204059834098 -0.19545789644298 -1.76642967664407]  x3=[0.1272140148953 20.8639593582677 21.0536785332865;314.159265358979 314.159265358979 314.159265358979;0.963303922847719 -0.182607459948898 -1.75383432614583]  x4=[0.105943954693919 28.7200541309178 28.911709925791;314.159265358979 314.159265358979 314.159265358979;1.06860599999645 -0.205774210364396 -1.77658577694556]  x5=5.31853471099837e-06  V1=ones(3,3)  V2=ones(3,3)  I1=ones(3,3)  I2=ones(3,3)  nHarmo=1  Measurements=None  Decoupling=off  VsMag0=0  VrMag0=0  VsAngle0=0  VrAngle0=0  IsMag0=0  IrMag0=0  IsAngle0=0  IrAngle0=0
      settings: SourceProductBaseCode=PS
  Line 161 : spsDistributedParametersLineLib/Distributed Parameters Line  Phases=3  Length=0.20999  Frequency=50  Resistance=[0.646656091154803 0.0486237908083191 0.0486712220507153;0.0486237908083191 0.646561225344642 0.0486237934466192;0.0486712220507153 0.0486237934466192 0.646656091154803]  Inductance=[0.00282448912315926 0.00133270803418135 0.00132951476746136;0.00133270803418135 0.00282479813276775 0.00133799988507366;0.00132951476746136 0.00133799988507366 0.00282448912315926]  Capacitance=[7.89543174552926e-09 -1.85986777702161e-09 -1.7901190036642e-09;-1.85986777702161e-09 7.82540023894543e-09 -1.8957321828871e-09;-1.7901190036642e-09 -1.8957321828871e-09 7.91264394645417e-09]  x1=[133.212956294541 9754.96187830579 9755.18157544786;314.159265358979 314.159265358979 314.159265358979;1.01328015992117 -0.19419027070932 -1.76516218823196]  x2=[133.212573899875 9755.01179303504 9755.23118833384;314.159265358979 314.159265358979 314.159265358979;1.01328286247121 -0.194196782972676 -1.76516869949485]  x3=[0.116922378837229 24.8244987723414 25.0157517062807;314.159265358979 314.159265358979 314.159265358979;1.02384694406819 -0.214695025310743 -1.78551667182588]  x4=[0.116012463519141 24.824653168512 25.0156173913907;314.159265358979 314.159265358979 314.159265358979;1.00231586232785 -0.173943291837286 -1.74506548322588]  x5=1.00616135492121e-06  V1=ones(3,3)  V2=ones(3,3)  I1=ones(3,3)  I2=ones(3,3)  nHarmo=1  Measurements=None  Decoupling=off  VsMag0=0  VrMag0=0  VsAngle0=0  VrAngle0=0  IsMag0=0  IrMag0=0  IsAngle0=0  IrAngle0=0
      settings: SourceProductBaseCode=PS
  Line 162 : spsDistributedParametersLineLib/Distributed Parameters Line  Phases=3  Length=0.23002  Frequency=50  Resistance=[0.476003738225748 0.351747138225748 0.351747138225748;0.351747138225748 0.476003738225748 0.351747138225748;0.351747138225748 0.351747138225748 0.476003738225748]  Inductance=[0.000705954362986426 0.000459934243504405 0.000459934243504405;0.000459934243504405 0.000705954362986426 0.000459934243504405;0.000459934243504405 0.000459934243504405 0.000705954362986426]  Capacitance=[5.7561313269996e-07 -1.37543883484145e-07 -1.37543912800485e-07;-1.37543883484145e-07 5.75613027339387e-07 -1.37543875208088e-07;-1.37543912800485e-07 -1.37543875208088e-07 5.75613005057695e-07]  x1=[6.41121035240704 9756.04833673178 9757.09582307649;314.159265358979 314.159265358979 314.159265358979;1.23654829814384 -0.113249676833805 -1.68407953914731]  x2=[6.41121853130672 9756.0528059405 9757.1002927644;314.159265358979 314.159265358979 314.159265358979;1.23654535216566 -0.113250413305099 -1.68408027561849]  x3=[0.0869246970111877 524.662719171084 524.719010584966;314.159265358979 314.159265358979 314.159265358979;1.23494950284623 -0.114207224504611 -1.68503708674364]  x4=[0.0869246970627532 524.66271926423 524.719010676642;314.159265358979 314.159265358979 314.159265358979;1.23654535185146 -0.113250413305214 -1.68408027561887]  x5=5.08443513939426e-06  V1=ones(3,3)  V2=ones(3,3)  I1=ones(3,3)  I2=ones(3,3)  nHarmo=1  Measurements=None  Decoupling=off  VsMag0=0  VrMag0=0  VsAngle0=0  VrAngle0=0  IsMag0=0  IrMag0=0  IsAngle0=0  IrAngle0=0
      settings: SourceProductBaseCode=PS
  Line 163 : spsDistributedParametersLineLib/Distributed Parameters Line  Phases=3  Length=0.28003  Frequency=50  Resistance=[0.646656091154803 0.0486237908083191 0.0486712220507153;0.0486237908083191 0.646561225344642 0.0486237934466192;0.0486712220507153 0.0486237934466192 0.646656091154803]  Inductance=[0.00282448912315926 0.00133270803418135 0.00132951476746136;0.00133270803418135 0.00282479813276775 0.00133799988507366;0.00132951476746136 0.00133799988507366 0.00282448912315926]  Capacitance=[7.89543174552926e-09 -1.85986777702161e-09 -1.7901190036642e-09;-1.85986777702161e-09 7.82540023894543e-09 -1.8957321828871e-09;-1.7901190036642e-09 -1.8957321828871e-09 7.91264394645417e-09]  x1=[132.813568055349 9776.53144272244 9775.93082299833;314.159265358979 314.159265358979 314.159265358979;1.06937235717575 2.25621076332786 -2.45592417372771]  x2=[132.813625527751 9776.5341567036 9775.93354168532;314.159265358979 314.159265358979 314.159265358979;1.06937216903921 2.25621041013962 -2.45592452988051]  x3=[0.116107450888346 24.8722628401162 25.0616957360563;314.159265358979 314.159265358979 314.159265358979;1.06813364096176 2.25521425797155 -2.45692155981627]  x4=[0.116108157656713 24.8722624164289 25.0616961663547;314.159265358979 314.159265358979 314.159265358979;1.07018933461467 2.25687200582387 -2.4552623725697]  x5=1.3417561037125e-06  V1=ones(3,3)  V2=ones(3,3)  I1=ones(3,3)  I2=ones(3,3)  nHarmo=1  Measurements=None  Decoupling=off  VsMag0=0  VrMag0=0  VsAngle0=0  VrAngle0=0  IsMag0=0  IrMag0=0  IsAngle0=0  IrAngle0=0
      settings: SourceProductBaseCode=PS
  Line 164 : spsDistributedParametersLineLib/Distributed Parameters Line  Phases=3  Length=0.24001  Frequency=50  Resistance=[0.646656091154803 0.0486237908083191 0.0486712220507153;0.0486237908083191 0.646561225344642 0.0486237934466192;0.0486712220507153 0.0486237934466192 0.646656091154803]  Inductance=[0.00282448912315926 0.00133270803418135 0.00132951476746136;0.00133270803418135 0.00282479813276775 0.00133799988507366;0.00132951476746136 0.00133799988507366 0.00282448912315926]  Capacitance=[7.89543174552926e-09 -1.85986777702161e-09 -1.7901190036642e-09;-1.85986777702161e-09 7.82540023894543e-09 -1.8957321828871e-09;-1.7901190036642e-09 -1.8957321828871e-09 7.91264394645417e-09]  x1=[133.194568647634 9755.50630399661 9755.72029349299;314.159265358979 314.159265358979 314.159265358979;1.013291361415 -0.194177442318529 -1.76514874592774]  x2=[133.212956294535 9754.96187830601 9755.18157544808;314.159265358979 314.159265358979 314.159265358979;1.0132349712491 -0.194226170141407 -1.76519812183777]  x3=[0.125328903820071 20.8669007143422 21.0521453667912;314.159265358979 314.159265358979 314.159265358979;0.653300386966526 -0.20413730960201 -1.77786346106024]  x4=[0.12373277020837 28.7732287501418 28.9713793874404;314.159265358979 314.159265358979 314.159265358979;1.37772142981487 -0.1872440455304 -1.75620034412187]  x5=1.1500013657538e-06  V1=ones(3,3)  V2=ones(3,3)  I1=ones(3,3)  I2=ones(3,3)  nHarmo=1  Measurements=None  Decoupling=off  VsMag0=0  VrMag0=0  VsAngle0=0  VrAngle0=0  IsMag0=0  IrMag0=0  IsAngle0=0  IrAngle0=0
      settings: SourceProductBaseCode=PS
  Line 165 : spsDistributedParametersLineLib/Distributed Parameters Line  Phases=3  Length=0.03  Frequency=50  Resistance=[0.476003738225748 0.351747138225748 0.351747138225748;0.351747138225748 0.476003738225748 0.351747138225748;0.351747138225748 0.351747138225748 0.476003738225748]  Inductance=[0.000705954362986426 0.000459934243504405 0.000459934243504405;0.000459934243504405 0.000705954362986426 0.000459934243504405;0.000459934243504405 0.000459934243504405 0.000705954362986426]  Capacitance=[5.7561313269996e-07 -1.37543883484145e-07 -1.37543912800485e-07;-1.37543883484145e-07 5.75613027339387e-07 -1.37543875208088e-07;-1.37543912800485e-07 -1.37543875208088e-07 5.75613005057695e-07]  x1=[6.50811897326202 9752.0600676398 9753.11034638649;314.159265358979 314.159265358979 314.159265358979;1.24665709942908 -0.112800147820591 -1.68362811465462]  x2=[6.50812001931151 9752.06022248131 9753.11050168674;314.159265358979 314.159265358979 314.159265358979;1.24665526071987 -0.112800173320141 -1.68362814028077]  x3=[0.0883531077860304 524.974601017085 525.031036242802;314.159265358979 314.159265358979 314.159265358979;1.24320839917228 -0.112989666873702 -1.683818189854]  x4=[0.0885498648929423 524.974537968928 525.031099249763;314.159265358979 314.159265358979 314.159265358979;1.24988817636641 -0.112735499150203 -1.68356290998775]  x5=6.63129528657629e-07  V1=ones(3,3)  V2=ones(3,3)  I1=ones(3,3)  I2=ones(3,3)  nHarmo=1  Measurements=None  Decoupling=off  VsMag0=0  VrMag0=0  VsAngle0=0  VrAngle0=0  IsMag0=0  IrMag0=0  IsAngle0=0  IrAngle0=0
      settings: SourceProductBaseCode=PS
  Line 166 : spsDistributedParametersLineLib/Distributed Parameters Line  Phases=3  Length=0.02  Frequency=50  Resistance=[0.646656091154803 0.0486237908083191 0.0486712220507153;0.0486237908083191 0.646561225344642 0.0486237934466192;0.0486712220507153 0.0486237934466192 0.646656091154803]  Inductance=[0.00282448912315926 0.00133270803418135 0.00132951476746136;0.00133270803418135 0.00282479813276775 0.00133799988507366;0.00132951476746136 0.00133799988507366 0.00282448912315926]  Capacitance=[7.89543174552926e-09 -1.85986777702161e-09 -1.7901190036642e-09;-1.85986777702161e-09 7.82540023894543e-09 -1.8957321828871e-09;-1.7901190036642e-09 -1.8957321828871e-09 7.91264394645417e-09]  x1=[133.194568647634 9755.50630399661 9755.72029349299;314.159265358979 314.159265358979 314.159265358979;1.01362253928828 -0.193914343249312 -1.76488539640684]  x2=[133.194603479211 9755.50129375496 9755.7152942657;314.159265358979 314.159265358979 314.159265358979;1.01362261681545 -0.193914386957979 -1.76488543853518]  x3=[0.117078609261743 24.5504642621137 24.7415691631414;314.159265358979 314.159265358979 314.159265358979;1.00725367015182 -0.186532289093317 -1.75756213857955]  x4=[0.115837241496129 25.1031024736904 25.2944332493692;314.159265358979 314.159265358979 314.159265358979;1.02002947267648 -0.201157577706208 -1.77207230594531]  x5=9.5829454252223e-08  V1=ones(3,3)  V2=ones(3,3)  I1=ones(3,3)  I2=ones(3,3)  nHarmo=1  Measurements=None  Decoupling=off  VsMag0=0  VrMag0=0  VsAngle0=0  VrAngle0=0  IsMag0=0  IrMag0=0  IsAngle0=0  IrAngle0=0
      settings: SourceProductBaseCode=PS
  Line 167 : spsDistributedParametersLineLib/Distributed Parameters Line  Phases=3  Length=0.50001  Frequency=50  Resistance=[0.646656091154803 0.0486237908083191 0.0486712220507153;0.0486237908083191 0.646561225344642 0.0486237934466192;0.0486712220507153 0.0486237934466192 0.646656091154803]  Inductance=[0.00282448912315926 0.00133270803418135 0.00132951476746136;0.00133270803418135 0.00282479813276775 0.00133799988507366;0.00132951476746136 0.00133799988507366 0.00282448912315926]  Capacitance=[7.89543174552926e-09 -1.85986777702161e-09 -1.7901190036642e-09;-1.85986777702161e-09 7.82540023894543e-09 -1.8957321828871e-09;-1.7901190036642e-09 -1.8957321828871e-09 7.91264394645417e-09]  x1=[133.155335063346 9756.76318303855 9756.96500336633;314.159265358979 314.159265358979 314.159265358979;1.01301576189175 -0.194385429818844 -1.76535571588858]  x2=[133.194568647634 9755.50630399661 9755.72029349299;314.159265358979 314.159265358979 314.159265358979;1.01289998717268 -0.19448836344937 -1.76545996303348]  x3=[0.126152461795232 20.5862897183801 20.7708422824375;314.159265358979 314.159265358979 314.159265358979;0.648451396592185 -0.196378346686945 -1.77021918070282]  x4=[0.123409749592341 29.0420200766586 29.2398066595206;314.159265358979 314.159265358979 314.159265358979;1.38519573410615 -0.193571692295889 -1.76250197536644]  x5=2.3957842710327e-06  V1=ones(3,3)  V2=ones(3,3)  I1=ones(3,3)  I2=ones(3,3)  nHarmo=1  Measurements=None  Decoupling=off  VsMag0=0  VrMag0=0  VsAngle0=0  VrAngle0=0  IsMag0=0  IrMag0=0  IsAngle0=0  IrAngle0=0
      settings: SourceProductBaseCode=PS
  Line 168 : spsDistributedParametersLineLib/Distributed Parameters Line  Phases=3  Length=1.11  Frequency=50  Resistance=[0.502970710632245 0.0486237908083191 0.0486712220507153;0.0486237908083191 0.502875844822084 0.0486237934466192;0.0486712220507153 0.0486237934466192 0.502970710632245]  Inductance=[0.00286900545038753 0.00133270803418135 0.00132951476746136;0.00133270803418135 0.00286931445999602 0.00133799988507366;0.00132951476746136 0.00133799988507366 0.00286900545038753]  Capacitance=[8.11484299003193e-09 -1.94249816214699e-09 -1.86930692621136e-09;-1.94249816214699e-09 8.0425699231653e-09 -1.98049571960044e-09;-1.86930692621136e-09 -1.98049571960044e-09 8.13337738722527e-09]  x1=[236.087449776743 9767.90155061693 9767.89086441013;314.159265358979 314.159265358979 314.159265358979;0.991851144829654 -0.188309772465034 -1.75930307769869]  x2=[236.087786385874 9767.91068514074 9767.90001949522;314.159265358979 314.159265358979 314.159265358979;0.991850652618039 -0.188310650267137 -1.75930396306194]  x3=[0.206976190234936 24.8474327192003 25.0381906631817;314.159265358979 314.159265358979 314.159265358979;0.990162242458215 -0.189677805456445 -1.76067265354465]  x4=[0.206976190314536 24.8474327267111 25.0381906708973;314.159265358979 314.159265358979 314.159265358979;0.991850652557373 -0.188310650267942 -1.75930396306341]  x5=5.37516004033389e-06  V1=ones(3,3)  V2=ones(3,3)  I1=ones(3,3)  I2=ones(3,3)  nHarmo=1  Measurements=None  Decoupling=off  VsMag0=0  VrMag0=0  VsAngle0=0  VrAngle0=0  IsMag0=0  IrMag0=0  IsAngle0=0  IrAngle0=0
      settings: SourceProductBaseCode=PS
  Line 169 : spsDistributedParametersLineLib/Distributed Parameters Line  Phases=3  Length=0.03  Frequency=50  Resistance=[0.476003738225748 0.351747138225748 0.351747138225748;0.351747138225748 0.476003738225748 0.351747138225748;0.351747138225748 0.351747138225748 0.476003738225748]  Inductance=[0.000705954362986426 0.000459934243504405 0.000459934243504405;0.000459934243504405 0.000705954362986426 0.000459934243504405;0.000459934243504405 0.000459934243504405 0.000705954362986426]  Capacitance=[5.7561313269996e-07 -1.37543883484145e-07 -1.37543912800485e-07;-1.37543883484145e-07 5.75613027339387e-07 -1.37543875208088e-07;-1.37543912800485e-07 -1.37543875208088e-07 5.75613005057695e-07]  x1=[5.99241921292997 9768.97324723457 9769.95352904082;314.159265358979 314.159265358979 314.159265358979;1.25209062286006 -0.111644187633337 -1.68246720928919]  x2=[5.99242018897739 9768.97340234458 9769.95368460924;314.159265358979 314.159265358979 314.159265358979;1.25208863094493 -0.111644213132886 -1.68246723491533]  x3=[0.0813429825296954 525.885074251493 525.937741218099;314.159265358979 314.159265358979 314.159265358979;1.24837137365515 -0.111833706676015 -1.68265728445941]  x4=[0.0815424486793567 525.885011101512 525.937804326849;314.159265358979 314.159265358979 314.159265358979;1.25559068564694 -0.111579538972857 -1.68240200465121]  x5=6.63129528657629e-07  V1=ones(3,3)  V2=ones(3,3)  I1=ones(3,3)  I2=ones(3,3)  nHarmo=1  Measurements=None  Decoupling=off  VsMag0=0  VrMag0=0  VsAngle0=0  VrAngle0=0  IsMag0=0  IrMag0=0  IsAngle0=0  IrAngle0=0
      settings: SourceProductBaseCode=PS
  Line 17 : spsDistributedParametersLineLib/Distributed Parameters Line  Phases=3  Length=0.20998  Frequency=50  Resistance=[0.646656091154803 0.0486237908083191 0.0486712220507153;0.0486237908083191 0.646561225344642 0.0486237934466192;0.0486712220507153 0.0486237934466192 0.646656091154803]  Inductance=[0.00282448912315926 0.00133270803418135 0.00132951476746136;0.00133270803418135 0.00282479813276775 0.00133799988507366;0.00132951476746136 0.00133799988507366 0.00282448912315926]  Capacitance=[7.89543174552926e-09 -1.85986777702161e-09 -1.7901190036642e-09;-1.85986777702161e-09 7.82540023894543e-09 -1.8957321828871e-09;-1.7901190036642e-09 -1.8957321828871e-09 7.91264394645417e-09]  x1=[131.767945414107 9846.34212093538 9845.8560497775;314.159265358979 314.159265358979 314.159265358979;1.06966778139996 2.25907396154742 -2.45306575464316]  x2=[131.76740411026 9846.39251981088 9845.90610397102;314.159265358979 314.159265358979 314.159265358979;1.06966830705476 2.25906745111642 -2.45307226700405]  x3=[0.114822168552034 25.057195498004 25.248133645087;314.159265358979 314.159265358979 314.159265358979;1.08111106989748 2.23856935288448 -2.47342039003085]  x4=[0.115587851307072 25.0570487145759 25.2482779199422;314.159265358979 314.159265358979 314.159265358979;1.05798577970981 2.27932105439622 -2.43296911117125]  x5=1.00611344019409e-06  V1=ones(3,3)  V2=ones(3,3)  I1=ones(3,3)  I2=ones(3,3)  nHarmo=1  Measurements=None  Decoupling=off  VsMag0=0  VrMag0=0  VsAngle0=0  VrAngle0=0  IsMag0=0  IrMag0=0  IsAngle0=0  IrAngle0=0
      settings: SourceProductBaseCode=PS
  Line 170 : spsDistributedParametersLineLib/Distributed Parameters Line  Phases=3  Length=0.28003  Frequency=50  Resistance=[0.476003738225748 0.351747138225748 0.351747138225748;0.351747138225748 0.476003738225748 0.351747138225748;0.351747138225748 0.351747138225748 0.476003738225748]  Inductance=[0.000705954362986426 0.000459934243504405 0.000459934243504405;0.000459934243504405 0.000705954362986426 0.000459934243504405;0.000459934243504405 0.000459934243504405 0.000705954362986426]  Capacitance=[5.7561313269996e-07 -1.37543883484145e-07 -1.37543912800485e-07;-1.37543883484145e-07 5.75613027339387e-07 -1.37543875208088e-07;-1.37543912800485e-07 -1.37543875208088e-07 5.75613005057695e-07]  x1=[5.99241921292997 9768.97324723457 9769.95352904082;314.159265358979 314.159265358979 314.159265358979;1.25035434548543 -0.112684634438584 -1.683507656014]  x2=[5.99135172723786 9768.62607576064 9769.60702568744;314.159265358979 314.159265358979 314.159265358979;1.24770931597226 -0.11270011011297 -1.68352337486112]  x3=[0.0724819414594343 516.092719039476 516.128312599108;314.159265358979 314.159265358979 314.159265358979;0.679064888621912 -0.11067965195896 -1.68161544111268]  x4=[0.108584481526385 534.343744664943 534.413224943926;314.159265358979 314.159265358979 314.159265358979;1.61594876283112 -0.115782266890483 -1.68649646510535]  x5=6.18987206366653e-06  V1=ones(3,3)  V2=ones(3,3)  I1=ones(3,3)  I2=ones(3,3)  nHarmo=1  Measurements=None  Decoupling=off  VsMag0=0  VrMag0=0  VsAngle0=0  VrAngle0=0  IsMag0=0  IrMag0=0  IsAngle0=0  IrAngle0=0
      settings: SourceProductBaseCode=PS
  Line 171 : spsDistributedParametersLineLib/Distributed Parameters Line  Phases=3  Length=0.28003  Frequency=50  Resistance=[0.646656091154803 0.0486237908083191 0.0486712220507153;0.0486237908083191 0.646561225344642 0.0486237934466192;0.0486712220507153 0.0486237934466192 0.646656091154803]  Inductance=[0.00282448912315926 0.00133270803418135 0.00132951476746136;0.00133270803418135 0.00282479813276775 0.00133799988507366;0.00132951476746136 0.00133799988507366 0.00282448912315926]  Capacitance=[7.89543174552926e-09 -1.85986777702161e-09 -1.7901190036642e-09;-1.85986777702161e-09 7.82540023894543e-09 -1.8957321828871e-09;-1.7901190036642e-09 -1.8957321828871e-09 7.91264394645417e-09]  x1=[132.951673972411 9767.59276382106 9767.73424363627;314.159265358979 314.159265358979 314.159265358979;1.01369261013533 -0.193522334632941 -1.76448884707882]  x2=[132.981049340391 9765.8433726981 9765.99330028453;314.159265358979 314.159265358979 314.159265358979;1.01365633170362 -0.193617226876779 -1.76458409425033]  x3=[0.141119141376538 15.7895146776316 15.9651119150445;314.159265358979 314.159265358979 314.159265358979;0.613078585455003 -0.0887869412105725 -1.6648175588106]  x4=[0.116347517312938 34.0321525445189 34.2283903852733;314.159265358979 314.159265358979 314.159265358979;1.50588380340396 -0.242359653275739 -1.81123339774317]  x5=1.3417561037125e-06  V1=ones(3,3)  V2=ones(3,3)  I1=ones(3,3)  I2=ones(3,3)  nHarmo=1  Measurements=None  Decoupling=off  VsMag0=0  VrMag0=0  VsAngle0=0  VrAngle0=0  IsMag0=0  IrMag0=0  IsAngle0=0  IrAngle0=0
      settings: SourceProductBaseCode=PS
  Line 172 : spsDistributedParametersLineLib/Distributed Parameters Line  Phases=3  Length=0.3  Frequency=50  Resistance=[0.80718830189013 0.0486237908083191 0.0486712220507153;0.0486237908083191 0.807093436079969 0.0486237934466192;0.0486712220507153 0.0486237934466192 0.80718830189013]  Inductance=[0.00279786707424938 0.00133270803418135 0.00132951476746136;0.00133270803418135 0.00279817608385787 0.00133799988507366;0.00132951476746136 0.00133799988507366 0.00279786707424938]  Capacitance=[7.73340098830622e-09 -1.79942827973291e-09 -1.73218055098733e-09;-1.79942827973291e-09 7.66505189233746e-09 -1.83375898618858e-09;-1.73218055098733e-09 -1.83375898618858e-09 7.749673531177e-09]  x1=[56.8282812943665 9765.9283516482 9766.16105782198;314.159265358979 314.159265358979 314.159265358979;1.08019932407203 -0.197945599694674 -1.76887290041001]  x2=[56.8282870029121 9765.92895491753 9766.16166212552;314.159265358979 314.159265358979 314.159265358979;1.08019927115132 -0.197945701193215 -1.76887300275379]  x3=[0.0495151193185665 24.7795380633146 24.9689321577629;314.159265358979 314.159265358979 314.159265358979;1.07975107316628 -0.198297141160986 -1.76922473926614]  x4=[0.049515119325593 24.7795380636081 24.968932158021;314.159265358979 314.159265358979 314.159265358979;1.0801992705363 -0.197945701193326 -1.76887300275506]  x5=1.42674452918375e-06  V1=ones(3,3)  V2=ones(3,3)  I1=ones(3,3)  I2=ones(3,3)  nHarmo=1  Measurements=None  Decoupling=off  VsMag0=0  VrMag0=0  VsAngle0=0  VrAngle0=0  IsMag0=0  IrMag0=0  IsAngle0=0  IrAngle0=0
      settings: SourceProductBaseCode=PS
  Line 173 : spsDistributedParametersLineLib/Distributed Parameters Line  Phases=3  Length=0.25999  Frequency=50  Resistance=[0.646656091154803 0.0486237908083191 0.0486712220507153;0.0486237908083191 0.646561225344642 0.0486237934466192;0.0486712220507153 0.0486237934466192 0.646656091154803]  Inductance=[0.00282448912315926 0.00133270803418135 0.00132951476746136;0.00133270803418135 0.00282479813276775 0.00133799988507366;0.00132951476746136 0.00133799988507366 0.00282448912315926]  Capacitance=[7.89543174552926e-09 -1.85986777702161e-09 -1.7901190036642e-09;-1.85986777702161e-09 7.82540023894543e-09 -1.8957321828871e-09;-1.7901190036642e-09 -1.8957321828871e-09 7.91264394645417e-09]  x1=[132.981049340391 9765.8433726981 9765.99330028453;314.159265358979 314.159265358979 314.159265358979;1.01368649762599 -0.193593262032694 -1.76456010659341]  x2=[133.008279258237 9764.21720820124 9764.37497580907;314.159265358979 314.159265358979 314.159265358979;1.01365296883468 -0.193681127423475 -1.76464829925623]  x3=[0.141106944750564 15.7870602259223 15.9625876697711;314.159265358979 314.159265358979 314.159265358979;0.613795007971786 -0.087810244009445 -1.66384472554151]  x4=[0.116323237051456 34.0296399897323 34.2258448412789;314.159265358979 314.159265358979 314.159265358979;1.50506468848456 -0.242887844498693 -1.81176305588595]  x5=1.24573499055177e-06  V1=ones(3,3)  V2=ones(3,3)  I1=ones(3,3)  I2=ones(3,3)  nHarmo=1  Measurements=None  Decoupling=off  VsMag0=0  VrMag0=0  VsAngle0=0  VrAngle0=0  IsMag0=0  IrMag0=0  IsAngle0=0  IrAngle0=0
      settings: SourceProductBaseCode=PS
  Line 174 : spsDistributedParametersLineLib/Distributed Parameters Line  Phases=3  Length=0.3  Frequency=50  Resistance=[0.80718830189013 0.0486237908083191 0.0486712220507153;0.0486237908083191 0.807093436079969 0.0486237934466192;0.0486712220507153 0.0486237934466192 0.80718830189013]  Inductance=[0.00279786707424938 0.00133270803418135 0.00132951476746136;0.00133270803418135 0.00279817608385787 0.00133799988507366;0.00132951476746136 0.00133799988507366 0.00279786707424938]  Capacitance=[7.73340098830622e-09 -1.79942827973291e-09 -1.73218055098733e-09;-1.79942827973291e-09 7.66505189233746e-09 -1.83375898618858e-09;-1.73218055098733e-09 -1.83375898618858e-09 7.749673531177e-09]  x1=[56.4359273308015 9776.6186320112 9776.10134751687;314.159265358979 314.159265358979 314.159265358979;1.03006205583648 2.26050537847559 -2.45166787257913]  x2=[56.4359329999779 9776.61923594089 9776.10195243551;314.159265358979 314.159265358979 314.159265358979;1.03006200291575 2.26050527697705 -2.45166797492291]  x3=[0.0491732569376031 24.8066630021609 24.9943462808698;314.159265358979 314.159265358979 314.159265358979;1.02961380363567 2.26015383701032 -2.45201971143809]  x4=[0.0491732568829387 24.8066630024403 24.9943462810512;314.159265358979 314.159265358979 314.159265358979;1.03006200364369 2.260505276976 -2.45166797492146]  x5=1.42674452918375e-06  V1=ones(3,3)  V2=ones(3,3)  I1=ones(3,3)  I2=ones(3,3)  nHarmo=1  Measurements=None  Decoupling=off  VsMag0=0  VrMag0=0  VsAngle0=0  VrAngle0=0  IsMag0=0  IrMag0=0  IsAngle0=0  IrAngle0=0
      settings: SourceProductBaseCode=PS
  Line 175 : spsDistributedParametersLineLib/Distributed Parameters Line  Phases=3  Length=0.02  Frequency=50  Resistance=[0.476003738225748 0.351747138225748 0.351747138225748;0.351747138225748 0.476003738225748 0.351747138225748;0.351747138225748 0.351747138225748 0.476003738225748]  Inductance=[0.000705954362986426 0.000459934243504405 0.000459934243504405;0.000459934243504405 0.000705954362986426 0.000459934243504405;0.000459934243504405 0.000459934243504405 0.000705954362986426]  Capacitance=[5.7561313269996e-07 -1.37543883484145e-07 -1.37543912800485e-07;-1.37543883484145e-07 5.75613027339387e-07 -1.37543875208088e-07;-1.37543912800485e-07 -1.37543875208088e-07 5.75613005057695e-07]  x1=[5.99249545666378 9769.00243083192 9769.9826650685;314.159265358979 314.159265358979 314.159265358979;1.2523506351562 -0.111601335421504 -1.68242433962915]  x2=[5.99241921292954 9768.97324723457 9769.95352904082;314.159265358979 314.159265358979 314.159265358979;1.25216006562189 -0.111602574754672 -1.68242559641374]  x3=[0.0727833016968537 515.264390015599 515.299740449999;314.159265358979 314.159265358979 314.159265358979;0.677319616402788 -0.10823982193766 -1.67917639728566]  x4=[0.109240609335364 536.565872770507 536.6356014464;314.159265358979 314.159265358979 314.159265358979;1.6228814826352 -0.114912188672962 -1.68562595381408]  x5=4.42086352438419e-07  V1=ones(3,3)  V2=ones(3,3)  I1=ones(3,3)  I2=ones(3,3)  nHarmo=1  Measurements=None  Decoupling=off  VsMag0=0  VrMag0=0  VsAngle0=0  VrAngle0=0  IsMag0=0  IrMag0=0  IsAngle0=0  IrAngle0=0
      settings: SourceProductBaseCode=PS
  Line 176 : spsDistributedParametersLineLib/Distributed Parameters Line  Phases=3  Length=1.7102  Frequency=50  Resistance=[0.646656091154803 0.0486237908083191 0.0486712220507153;0.0486237908083191 0.646561225344642 0.0486237934466192;0.0486712220507153 0.0486237934466192 0.646656091154803]  Inductance=[0.00282448912315926 0.00133270803418135 0.00132951476746136;0.00133270803418135 0.00282479813276775 0.00133799988507366;0.00132951476746136 0.00133799988507366 0.00282448912315926]  Capacitance=[7.89543174552926e-09 -1.85986777702161e-09 -1.7901190036642e-09;-1.85986777702161e-09 7.82540023894543e-09 -1.8957321828871e-09;-1.7901190036642e-09 -1.8957321828871e-09 7.91264394645417e-09]  x1=[132.762640557686 9780.24311209195 9780.33092876166;314.159265358979 314.159265358979 314.159265358979;1.01183193746653 -0.19451883723924 -1.76548526045289]  x2=[132.953702150468 9767.96925137807 9768.10961576044;314.159265358979 314.159265358979 314.159265358979;1.01168165905594 -0.195215880583077 -1.76618377309279]  x3=[0.145595992083632 14.2981187380914 14.4717038959328;314.159265358979 314.159265358979 314.159265358979;0.607335766162864 -0.0760898804976545 -1.65287508859505]  x4=[0.113609564243812 35.4966159500068 35.6924738465075;314.159265358979 314.159265358979 314.159265358979;1.53725109581476 -0.244049560446732 -1.81299005488765]  x5=8.19437663310758e-06  V1=ones(3,3)  V2=ones(3,3)  I1=ones(3,3)  I2=ones(3,3)  nHarmo=1  Measurements=None  Decoupling=off  VsMag0=0  VrMag0=0  VsAngle0=0  VrAngle0=0  IsMag0=0  IrMag0=0  IsAngle0=0  IrAngle0=0
      settings: SourceProductBaseCode=PS
  Line 177 : spsDistributedParametersLineLib/Distributed Parameters Line  Phases=3  Length=0.02  Frequency=50  Resistance=[0.646656091154803 0.0486237908083191 0.0486712220507153;0.0486237908083191 0.646561225344642 0.0486237934466192;0.0486712220507153 0.0486237934466192 0.646656091154803]  Inductance=[0.00282448912315926 0.00133270803418135 0.00132951476746136;0.00133270803418135 0.00282479813276775 0.00133799988507366;0.00132951476746136 0.00133799988507366 0.00282448912315926]  Capacitance=[7.89543174552926e-09 -1.85986777702161e-09 -1.7901190036642e-09;-1.85986777702161e-09 7.82540023894543e-09 -1.8957321828871e-09;-1.7901190036642e-09 -1.8957321828871e-09 7.91264394645417e-09]  x1=[132.762640557686 9780.24311209195 9780.33092876166;314.159265358979 314.159265358979 314.159265358979;1.01437617109871 -0.192497610718672 -1.7634621098678]  x2=[132.762720707447 9780.23049526817 9780.3183253444;314.159265358979 314.159265358979 314.159265358979;1.0143766353958 -0.192498234836727 -1.76346272874598]  x3=[0.118441044312063 23.989642186314 24.1807738631193;314.159265358979 314.159265358979 314.159265358979;1.003286182108 -0.184294502015171 -1.75533298293138]  x4=[0.113729630600938 25.7900423988543 25.9816614845241;314.159265358979 314.159265358979 314.159265358979;1.02589534282753 -0.200151734355955 -1.77105147264792]  x5=9.5829454252223e-08  V1=ones(3,3)  V2=ones(3,3)  I1=ones(3,3)  I2=ones(3,3)  nHarmo=1  Measurements=None  Decoupling=off  VsMag0=0  VrMag0=0  VsAngle0=0  VrAngle0=0  IsMag0=0  IrMag0=0  IsAngle0=0  IrAngle0=0
      settings: SourceProductBaseCode=PS
